simulink model "tutorial_picooz_acquire_extmode"  (R2025b)
settings: Solver=FixedStepDiscrete  StartTime=0.0  StopTime=60  FixedStep=0.001  RelTol=1e-3  EnableMultiTasking=on
undefined symbols (not defined in the file or in its folder): A0, ADC, D10, H0, Max, MaxPer, ms, ns, P1, P113, P59, Pin, PWM3_Trg1, Resol, us
libraries: MCHP_Blockset x8, simulink x5, dspsrcs4 x1, dspstat3 x1
(part 1 of 2)
settings Model: SimulationMode=external  ExtModeTrigDuration=20  Creator=Lubin Kerhuel  LastModifiedBy=Lubin Kerhuel
settings OptimizationCC: DefaultParameterBehavior=Inlined  DefaultUnderspecifiedDataType=single  EnhancedBackFolding=on  BooleansAsBitfields=on  PassReuseOutputArgsAs=Individual arguments  ZeroExternalMemoryAtStartup=off  ZeroInternalMemoryAtStartup=off  OptimizeBlockOrder=speed  DifferentSizesBufferReuse=on  EfficientTunableParamExpr=on
settings DebuggingCC: ParameterTunabilityLossMsg=error
settings HardwareCC: ProdBitPerPointer=32.0  ProdBitPerSizeT=32.0  ProdBitPerPtrDiffT=32.0  ProdLargestAtomicInteger=Long  ProdWordSize=32.0  ProdLongLongMode=on  ProdHWDeviceType=Generic->Custom
settings ModelReferenceCC: ModelReferenceNumInstancesAllowed=Single
settings SFSimCC: MATLABDynamicMemAlloc=off
settings RTWCC: SystemTargetFile=MCHP_dsPIC33A_noTMF_stf.tlc  TLCOptions="-aExtModeXCPClassicInterface=0  -aCreateExtModeTypes=1 -aExtModeXCPSimulationTimeInTicks=1"  TemplateMakefile=MCHP_dsPIC33A.tmf  Toolchain=MPLAB XC-DSC - v4.00_TC1 for dsPIC DSCs (Microchip)  BuildConfiguration=Specify  Description=Microchip Embedded Target dsPIC33A no TMF (real-time)
settings CodeAppCC: ForceParamTrailComments=on  IgnoreCustomStorageClasses=off  MaxIdLength=255.0  OperatorAnnotations=on  SimulinkDataObjDesc=on  SFDataObjDesc=on  InsertBlockDesc=on
settings STFCustomTargetCC: SystemTargetFile=MCHP_dsPIC33A_noTMF_stf.tlc  TargetLangStandard=C99 (ISO)  MultiwordLength=256.0  ConcurrentExecutionCompliant=off  CombineOutputUpdateFcns=on  CombineSignalStateStructs=on  ERTCustomFileBanners=on  SupportContinuousTime=off  RemoveResetFunc=on  MATLABClassNameForMDSCustomization=Simulink.SoftwareTarget.ERTCustomization  GRTInterface=off  UseToolchainInfoCompliant=on  MCHP_AUTO_FLASH=off  LINKER_SCRIPT=p33AK512MPS512.gld  EXTMODE_DATA_UPLOAD=on  RTWGenSettings_txt="s.RefMasterBlk='PICOOZ_OL_ExtMode_Curiosity_dsPIC33AK512MPS512/Microchip Master';s.ChipIdN='[33  512  512]';s.ChipIdL1='AK';s.ChipIdL2='MPS';s.ChipIdL3=' ';s.arch3='33A';s.ChipId='33AK512MPS512';s.Arch='8';s.bitFieldsSFR='4';s.ChipRAM='32768';s.ChipRAM_XBegin='16384';s.ChipRAM_dma='[-1 -1]';s.FuseConfigTxt='#pragma config FICD_JTAGEN = OFF\\\\n';s.TimeStep_Timer='-1';s.TimeStep_SyncADC='1';s.ADPCFG='0';s.ANSEL_Exist='1';s.ANSEL='[-1 -1 -1 -1 -1 -1 -1 -1 -1 -1 -1]';s.TRIS='[65535  65535    255  65535     -1     -1     -1  65535     -1     -1     -1     -1     -1     -1     -1     -1     -1     -1     -1     -1     -1     -1     -1     -1     -1     -1     -1     -1     -1     -1     -1     -1     -1     -1     -1     -1     -1     -1     -1     -1     -1     -1     -1     -1     -1     -1     -1     -1     -1     -1     -1     -1     -1     -1     -1     -1     -1]';s.RPOR='[-1  -1  -1  -1  -1  -1  -1  -1  -1  -1  -1  -1  -1  -1  -1  -1  -1  -1  -1  -1  -1  -1  -1  -1  -1  -1  -1  -1  19  -1  -1  -1  -1  -1  -1  -1]';s.RPINR='[-1  -1  -1  -1  -1  -1  -1  -1  -1  -1  -1  -1  -1  59  -1  -1  -1  -1  -1  -1  -1  -1  -1  -1  -1  -1  -1  -1]';s.LATSET='[-1 -1 -1 -1 -1 -1 -1 -1 -1 -1 -1 -1 -1 -1 -1 -1 -1 -1 -1 -1 -1 -1 -1 -1 -1 -1 -1 -1 -1 -1 -1 -1 -1 -1 -1 -1 -1 -1 -1 -1 -1 -1 -1 -1 -1 -1 -1 -1 -1 -1 -1 -1 -1 -1 -1 -1 -1]';s.LATCLR='[-1 -1 -1 -1 -1 -1 -1 -1 -1 -1 -1 -1 -1 -1 -1 -1 -1 -1 -1 -1 -1 -1 -1 -1 -1 -1 -1 -1 -1 -1 -1 -1 -1 -1 -1 -1 -1 -1 -1 -1 -1 -1 -1 -1 -1 -1 -1 -1 -1 -1 -1 -1 -1 -1 -1 -1 -1]';s.ODC='[-1 -1 -1 -1 -1 -1 -1 -1 -1 -1 -1 -1 -1 -1 -1 -1 -1 -1 -1 -1 -1 -1 -1 -1 -1 -1 -1 -1 -1 -1 -1 -1 -1 -1 -1 -1 -1 -1 -1 -1 -1 -1 -1 -1 -1 -1 -1 -1 -1 -1 -1 -1 -1 -1 -1 -1 -1]';s.CNPU='[-1 -1 -1 -1 -1 -1 -1 -1 -1 -1 -1 -1 -1 -1 -1 -1 -1 -1 -1 -1 -1 -1 -1 -1 -1 -1 -1 -1 -1 -1 -1 -1 -1 -1 -1 -1 -1 -1 -1 -1 -1 -1 -1 -1 -1 -1 -1 -1 -1 -1 -1 -1 -1 -1 -1 -1 -1]';s.CNPD='[-1 -1 -1 -1 -1 -1 -1 -1 -1 -1 -1 -1 -1 -1 -1 -1 -1 -1 -1 -1 -1 -1 -1 -1 -1 -1 -1 -1 -1 -1 -1 -1 -1 -1 -1 -1 -1 -1 -1 -1 -1 -1 -1 -1 -1 -1 -1 -1 -1 -1 -1 -1 -1 -1 -1 -1 -1]';s.PortConfigTxt=' ';s.CLKDIV='0';s.PLLFBD='-1';s.PLLDIV='16815713';s.QUARTZ='8000000';s.SWITCH_OSC='16386';s.PLLRNG='-1';s.MASTER_BusyFlag='-1';s.POWERSAVE='0';s.MIPS='200000000';s.FLASH_ECC='0';s.PBxDIV='[-1]';s.CLKx_INTDIV='[-1 -1 -1 -1  0  1  0  0  0 -1 -1  0  0]';s.CLKx_FRACDIV='[-1   -1   -1   -1    0  256    0    0    0   -1   -1    0    0]';s.AN_type2='1';s.ACLKCON_reg='-1';s.nTIMERS='3';s.nSCCP='9';s.DOS_04094_cpu_33a_v1_dspic33a='1';s.DOS_04436_perseus_dspic33a='0';s.DOS_04928_gpio_ports_upb_v2_dspic33a='1';s.DOS_02672_math_progcrc_upb_v1_dspic33a='1';s.DOS_04993_sec_32bit_cp_upb_v1_dspic33a='1';s.DOS_03459_adc_pc_ctrl_upb_v2_dspic33a='0';s.DOS_04302_pwm_pc_upb_v3_dspic33a='0';s.DOS_03076_uart_protocol_upb_v1_dspic33a='1';s.DOS_01482_spi_i2s_upb_v1_dspic33a='1';s.DOS_05155_i2c_upb_v4_dspic33a='1';s.DOS_02359_sent_j2716_upb_v1_dspic33a='1';s.DOS_05177_qei_32b_upb_v2_dspic33a='1';s.DOS_01512_ccp_mccp_upb_v1_dspic33a='1';s.DOS_03496_dac_pdm_nbit_upb_v2_dspic33a='0';s.DOS_02673_tmr_classa_upb_v1_dspic33a='1';s.DOS_04776_perf_mon_upb_v1_dspic33a='1';s.DOS_03680_pfm_pbu_33a_upb_v1_dspic33a='1';s.DOS_04649_sec_pac_upb_v0_dspic33a='0';s.DOS_03966_io_integrity_monitor_upb_v1_dspic33a='1';s.DOS_04641_biss_master_upb_v1_dspic33a='1';s.DOS_04077_dma_upb_v1_dspic33a='1';s.DOS_04549_nvm_ctrl_32bit_upb_v1_dspic33a='1';s.DOS_04449_clk_cru_33a_upb_v1_dspic33a='1';s.DOS_03850_clk_monitor_upb_v1_dspic33a='1';s.DOS_04342_osc_rc8mhz_ctrl_upb_v4_dspic33a='1';s.DOS_04650_wdt_upb_v4_dspic33a='1';s.DOS_05178_ptg_pc_upb_v2_dspic33a='1';s.DOS_04181_data_ram_ctrl_upb_v1_dspic33a='1';s.DOS_04735_wdt_dmt_upb_v6_dspic33a='1';s.DOS_01577_cla_clc_upb_v1_dspic33a='1';s.DOS_03516_pwr_sib_upb_v3_dspic33a='0';s.DOS_03495_amp_pad_opamp_ctrl_upb_v2_dspic33a='1';s.DOS_05830_blueRidge_dspic33a='0';s.DOS_05972_adc_12b_upb_v3_itc_dspic33a='0';s.DOS_05404_adc_pc_ctrl_upb_v3_dspic33a='1';s.DOS_05226_pwm_pc_upb_v4_dspic33a='1';s.DOS_05514_qei_32b_upb_v3_dspic33a='0';s.DOS_05431_dac_pdm_nbit_upb_v3_dspic33a='1';s.DOS_05828_pfm_pbu_33a_upb_v2_dspic33a='0';s.DOS_05765_math_rdc_upb_v1_32bit='0';s.DOS_05908_math_cic_upb_v2_32bit='0';s.DOS_05801_dma_upb_v2_dspic33a='0';s.DOS_05461_pwr_sib_upb_v4_dspic33a='1';s.DOS_05420_amp_vref_ctl_upb_v1_dspic33a='1';s.DOS_05592_pwr_monitor_sib_upb_v1='0';s.DOS_05924_bus_dual_die_upb_v2='0';s.DOS_06048_sec_cam_v3_dspic33a='0';s.DOS_05922_i3c_upb_v1_32bit='0';s.DOS_06006_adc_soft_code_seq_v2_dspic33a='0';s.DOS_05442_icd_trace_33a_v1_dspic33a='0';s.DOS_04537_can_fd_upb_v3_dspic33a='1';s.DOS_05308_pegasus_dspic33a='1';s.DOS_02976_adc_12b_upb_v2_dspic33a='1';s.DOS_05226_apwm_pc_upb_v4_dspic33a='1';s.DOS_04649_sec_pac_upb_v1_dspic33a='1';s.DOS_05346_sec_cam_v2_dspic33a='1';s.DOS_03267_adc_soft_code_seq_v1_dspic33a='1';s.DOS_05557_serpens_dspic33a='0';s.DOS_05972_adc_12b_upb_v3_adc_dspic33a='0';s.DOS_03681_bmx_33a_upb_v1_dspic33a='0';s.DOS_02050_tmr_rtcc_upb_v1_dspic33a='0';s.DOS_04649_sec_pac_upb_serpens_dspic33a='0';s.DOS_05692_pwr_sib_upb_v5_dspic33a='0';s.DOS_06006_adc_soft_code_seq_v2_adc_dspic33a='0';s.DOS_02551_cpu_16bit_v7='0';s.DOS_01520_wdt_dmt_upb_v1_16bit='0';s.DOS_02359a_sent_j2716_upb_v1='0';s.DOS_02672_math_progcrc_upb_v1_16bit='0';s.DOS_01577_cla_clc_upb_v1='0';s.DOS_02915_ecc_v2='0';s.DOS_02673_tmr_classa_upb_v1_16bit='0';s.DOS_01494_qei_32b_upb_v1_16bit='0';s.DOS_02472_ppi_pmp16_upb_v1_16bit='0';s.DOS_01441_i2c_upb_v1_16bit_TLAH='0';s.DOS_03076_uart_protocol_upb_v1_16bit='0';s.DOS_01482='0';s.DOS_01483_pwm_16bit='0';s.DOS_02949_WACG='0';s.DOS_02316_nvm_ctrl_v1_16bit='0';s.DOS_03349_amp_pad_opamp_ctrl_upb_v1='0';s.DOS_02653_afe_current_bias_ctrl_upb_v1_16bit='0';s.DOS_01459_ptg_pc_upb_v1_16bit='0';s.DOS_01512_ccp_mccp_upb_v1_16bit='0';s.DOS_02519_dma_sfr_16bit_v2='0';s.DOS_02508c11='0';s.DOS_02475_dac_pdm_nbit_upb_v1_16bit='0';s.DOS_02467_gpio_upb_v1_16bit='0';s.DOS_00805_rst_integration_v4='0';s.DOS_02659_clk_sib_v12='0';s.DOS_02237_osc_dco_ctrl_upb_v1_16bit='0';s.DOS_02674_wdt_upb_v1_16bit='0';s.DOS_01407='0';s.DOS_03247_CAN_FD_UPB_V2_16_bit='0';s.DOS_03994_WAC07='0';s.DOS_02552_msi_upb_v1_Master='0';s.DOS_03667_pwm_pc_upb_v2_16bit='0';s.DOS_04180_drm_ctrl_ecc_v1='0';s.DOS_03431_STX03='0';s.DOS_03516_pwr_sib_upb_v3='0';s.DOS_02552_msi_upb_v1_Slave='0';s.DOS_04621_amp_pga_ctrl_upb_v3='0';s.DOS_02497_WACV='0';s.DOS_02593_amp_pga_ctrl_pb_v2_16bit='0';s.DOS_01461_afe_ctmu_con_upb_v1_16bit='0';s.DOS_02497_WACA='0';s.DOS_02478_uart_irda_upb_v1_16bit='0';s.DOS_00929='0';s.DOS_01198='0';s.DOS_03029_WACH='0';s.DOS_01483_apwm_16bit='0';s.DOS_04797_WAC0A='0';s.DOS_04884_WAC0B='0';s.DOS_04797_WAC09='0';s.DOS_03662_WACU='0';s.DOS_00794='0';s.DOS_00931='0';s.DOS_00932='0';s.DOS_00942='0';s.DOS_00938='0';s.DOS_00996='0';s.DOS_00997='0';s.DOS_00998='0';s.DOS_00209='0';s.DOS_01555_adc='0';s.DOS_01293='0';s.DOS_00828='0';s.DOS_01116='0';s.DOS_01017_RPORx='0';s.DOS_01017_RPINRx='0';s.DOS_01555_nvm_tsmc18_v2_16bit='0';s.DOS_00804='0';s.DOS_00826='0';s.DOS_01555_TLAK_PMDx='0';s.DOS_01555_TLAK_INT_='0';s.DOS_00933='0';s.DOS_01555='0';s.DOS_01555_ptg='0';s.DOS_00958='0';s.DOS_01117_PORTx='0';s.DOS_00999='0';s.DOS_01041='0';s.DOS_00892='0';s.DOS_01287_TLAC_PMDx='0';s.DOS_01287_TLAC_INT_='0';s.DOS_01424='0';s.DOS_01332='0';s.DOS_01468_PMBA_current_source='0';s.DOS_02291_PGA='0';s.DOS_01467_Comparator='0';s.DOS_01498_TLAY='0';s.DOS_00993_PLL_120MHz='0';s.DOS_01332_ptg_pc_v1='0';s.DOS_00958_pwm_TLAY='0';s.TLAY_IOPorts='0';s.DOS_00929q='0';s.DOS_02415_spi_v5='0';s.DOS_RPINRx_16bit_2='0';s.DOS_01497_TLAH_PMDx='0';s.DOS_02550_TLAL_INT='0';s.DOS_00958_pwm_TLAH='0';s.DOS_01287_TLAH_INT_='0';s.DOS_01113='0';s.DOS_01017_PMDx='0';s.DOS_00927='0';s.DOS_01080='0';s.DOS_00794_cpu_16bit_v3='0';s.DOS_02192_TLCD_PMDx='0';s.DOS_02192_TLCD_INT_='0';s.DOS_02192_cmp='0';s.DOS_00958_pwm_TLCD='0';s.DOS_02192_PORTx_TLCD='0';s.DOS_00936='0';s.DOS_00995='0';s.DOS_00546='0';s.DOS_00474='0';s.DOS_02481_WACP_Config='0';s.DOS_03088_pfm_cache_ocp_v2_WACK='0';s.DOS_02819_pfm_ctrl_32bit_upb_v2='0';s.DOS_02674_wdt_upb_v1_32bit='0';s.DOS_01520_wdt_dmt_upb_v1='0';s.DOS_02869_icd_jtag_bvci_upb_v2='0';s.DOS_02823_WACJ_clk_cru_upb_v2='0';s.DOS_02823_WACN_clk_cru_upb_v2='0';s.DOS_01423_RPINRx='0';s.DOS_02481_RPORx='0';s.DOS_02511_pwr_sib_upb_v1_32bit='0';s.DOS_02907_WACP_int_evic_v3='0';s.DOS_01500_dma_bvci_v2='0';s.DOS_02141_tmr_classa_pb_v2='0';s.DOS_02815_tmr_classb_upb_v1='0';s.DOS_00740_icap_pb_v1='0';s.DOS_00749_ocmp_pb_v1='0';s.DOS_01441_i2c_upb_v1_32bit='0';s.DOS_01329_spi_pb_v2='0';s.DOS_02478_uart_irda_upb_v1_32bit='0';s.DOS_01477_pwm_mc_upb_v1='0';s.DOS_01494_qei_32b_upb_v1='0';s.DOS_03554_cmp_control_upb_v2_32bit='0';s.DOS_01445_dac_nbit__control_upb_v1_32bit='0';s.DOS_01461_afe_ctmu_con_upb_v1='0';s.DOS_01577_cla_clc_upb_v1_32bit='0';s.DOS_02467_gpio_ports_upb_v1='0';s.DOS_02508_WACP_adc_sar_ctrl_upb_v1='0';s.DOS_01261_tmr_rtcc_WACJ_K_N_P_pb_v2='0';s.DOS_EIP_00136_ssx_v1='0';s.DOS_02481_WACK_MC_Config='0';s.DOS_02907_WACN_GP_int_evic_v3='0';s.DOS_02508_adc_sar_ctrl_upb_v1_PIC32MK='0';s.DOS_01261_tmr_rtcc_pb_v2='0';s.DOS_01475_lpwr_deep_sleep_ctrl_v2='0';s.DOS_02907_WACN_MC_int_evic_v3='0';s.DOS_03247_can_fd_upb_v2_pic32mk='0';s.DOS_02907_WACK_MC_int_evic_v3='0';s.DOS_02514_dfm_strl_sst_upb_v1='0';s.DOS_02472_ppi_pmp16_upb_v1='0';s.DOS_02813a_usb_otgcore_pb_v3='0';s.DOS_02481_WACJ_MC_Config='0';s.DOS_02569_pfm_cache_ocp_v1='0';s.DOS_02481_WACJ_MC_int_evic_v3='0';s.DOS_01459_ptg_pc_upb_v1_SIC='0';s.DOS_01427_cmp_control_upb_v1_32bit='0';s.DOS_01152_can_bvci_v1='0';s.DOS_02787_WACD_Config='0';s.DOS_00800_dac_4bit_ctrl_pb_v1='0';s.DOS_01539_icd_jtag_pb_v2='0';s.DOS_02823_clk_cru_upb_v2='0';s.DOS_01423_RPORx='0';s.DOS_02907_WACD_int_evic_v3='0';s.DOS_00734_uart_irda_pb_v1='0';s.DOS_00687_tmr_classa_pb_v1='0';s.DOS_00745_tmr_classb_pb_v1='0';s.DOS_02508_adc_sar_ctrl_upb_v1='0';s.DOS_00866_cmp_control_pb_v2='0';s.DOS_01114_eth_bvci_v1='0';s.DOS_02831_usb_clk_rst_v2='0';s.DOS_01643_pfm_cache_ahb_v2='0';s.DOS_EIP_00206r5_sqi_v2='0';s.DOS_EIP_00124_usb_hs_otgcore_v1='0';s.DOS_EIP_00218_math_rng_ahbs_v2='0';s.DOS_EIP_00109_ebi_v1='0';s.DOS_EIP_00158_crypto_v1='0';s.UART_TX_IMPLEMENTATION='[2]';s.UART_RX_IMPLEMENTATION='[2]';s.UART_TX_DMACHANNEL='[0]';s.UART_HALF_DUPLEX_MODE='[0]';s.UART_TX_THREAD_PROTECTION='[9]';"  HOST_PLATFORM=PC  PIC_REF=33AK512MPS512  OBJDUMP=xc-dsc-objdump  BIN2HEX=xc-dsc-bin2hex  MCHP_MULTITHREAD_COMPILATION=on  TIMER_START="[0  0  0  0]"  LinkWithMaster=off  GCCPATH=C:/PROGRA~1/MICROC~1/xc-dsc/V44CDE~1.00_/bin  AssemblyListing=off  AR1=xc-dsc-ar  OPTIM_GCC=-O2 -fno-short-double -mno-eds-warn -mconst-in-data -mlarge-data -mlarge-aggregate -g -Wa,--reorder  LDFLAGS='--report-mem,-Map=$(PRODUCT_NAME).map,-cref,-lq-dsp'  ProduceHexOutput=off  TIMER_PERIOD="[0      0      0  65535]"  GCC1=xc-dsc-gcc.exe  TIMER_PRESCALER="[-1 -1 -1  3 -1 -1 -1 -1 -1 -1 -1 -1]"  MCHP_XCP_MemoryBlockParameters=[-1 8]
settings ERTTargetCC: ExtMode=on  ExtModeTransport=1.0  ExtModeStaticAlloc=on  ExtModeMaxTrigDuration=20.0  ExtModeStaticAllocSize=2048.0  ExtModeMexFile=ext_xcp  ExtModeMexArgs=1 27 460800 './PICOOZ_OL_ExtMode_Curiosity_dsPIC33AK512MPS512.X/PICOOZ_OL_ExtMode_Curiosity_dsPIC33AK512MPS512.elf'  ExtModeIntrfLevel=Level2 - Open  ERTSrcFileBannerTemplate=MCHP_dsPIC_code_template.cgt  ERTHdrFileBannerTemplate=MCHP_dsPIC_code_template.cgt  ERTDataSrcFileTemplate=MCHP_dsPIC_code_template.cgt  ERTDataHdrFileTemplate=MCHP_dsPIC_code_template.cgt  ERTCustomFileTemplate=MCHP_main.tlc  MaxLineWidth=110.0  TargetLangStandard=C99 (ISO)  ParMdlRefBuildCompliant=off  CompOptLevelCompliant=off  ConcurrentExecutionCompliant=off  CombineSignalStateStructs=on  SupportNonInlinedSFcns=on  ModelStepFunctionPrototypeControlCompliant=off  CPPClassGenCompliant=off

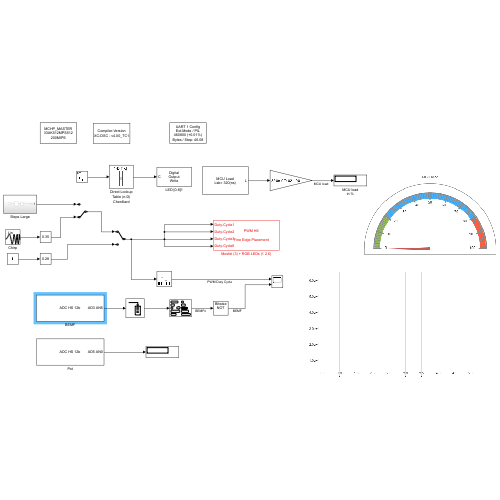
[thumbnail: Simulink's stored preview of the top-level diagram]
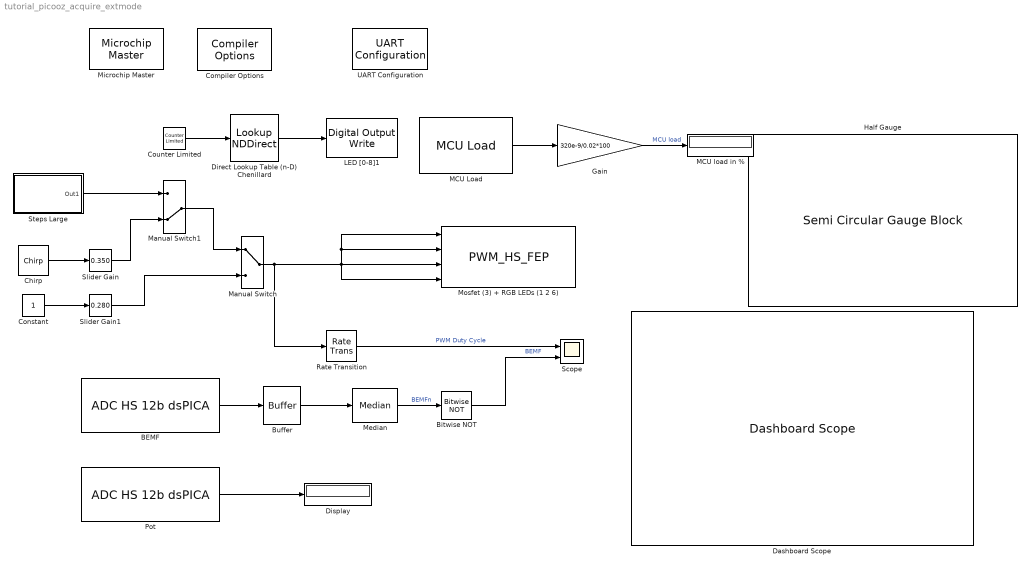
== system tutorial_picooz_acquire_extmode ==
  BEMF : MCHP_Blockset/Analog IO/ADC HS 12b dsPICA  ADCREF=ADC 1 and ADC 2  ADC1_refChannel=Not used  ADC2_refChannel=Not used  ADC3_refChannel=0 (highest priority)  ADC4_refChannel=Not used  ADC5_refChannel=Not used  CALRATE=once at startup  VREF_RNG=3.0V to 3.6V  BUFEN=off  info=0  SampleTime=.001  MCHP_PORT={ADC1_seq0.0}{ADC1A2}15:2:A2;{ADC2_seq0.0}{ADC2B0}15:2:B0;{ADC1_seq1.0}{ADC1A2}15:2:A2;{ADC2_seq1.0}{ADC2B0}15:2:B0;{ADC1_seq2.0}{ADC1A2}15:2:A2;{ADC2_seq2.0}{ADC2B0}15:2:B0;{ADC1_seq3.0}{ADC1A2}15:2:A2;{ADC2_seq3.0}{ADC2B0}15:2:B0;{ADC1_seq4.0}{ADC1A2}15:2:A2;{ADC2_seq4.0}{ADC2B0}15:2:B0;{ADC1_seq5.0}{ADC1A2}15:2:A2;{ADC2_seq5.0}{ADC2B0}15:2:B0;{ADC1_seq0.0}{ADC1A2}15:2:A2;{ADC2_seq0.0}{ADC2B0}15:2:B0;{ADC1_seq1.0}{ADC1A2}15:2:A2;{ADC2_seq1.0}{ADC2B0}15:2:B0;{ADC1_seq2.0}{ADC1A2}15:2:A2;{ADC2_seq2.0}{ADC2B0}15:2:B0;{ADC1_seq3.0}{ADC1A2}15:2:A2;{ADC2_seq3.0}{ADC2B0}15:2:B0;{ADC1_seq4.0}{ADC1A2}15:2:A2;{ADC2_seq4.0}{ADC2B0}15:2:B0;{ADC1_seq5.0}{ADC1A2}15:2:A2;{ADC2_seq5.0}{ADC2B0}15:2:B0;  MCHP_MASTERLINK=PICOOZ_OL_ExtMode_Curiosity_dsPIC33AK512MPS512/Microchip Master  MCHP_CRC=27486782  ADC_Synchronisation=Triggered by custom source  ADC_Trig_TXT=PWM3_Trg1  ADC_TrigTimeStep=on  TrigSource_seq0_TXT=PWM3 adc trig 1  SampleTime_seq0_Tad_TXT="4.5 Tad  = 56.2ns  -  Rin < 5.2 kOhm"  ADC1_seq0_TXT=AD1 AN0 / A2 / Pin[25]  ADC1_seq0_align=Left aligned  ADC1_seq0_overSampling=x1 (12 bits)  ADC2_seq0_TXT=AD2 AN0 / B0 / Pin[41]  ADC2_seq0_align=Right aligned  ADC2_seq0_overSampling=x1 (12 bits)  ADC3_seq0_TXT=AD3 AN5 / A0 / Pin[4]  ADC3_seq0_align=Left aligned  ADC3_seq0_overSampling=x256 (16 bits)  ADC4_seq0_TXT=AD4 AN0 / B4 / Pin[57]  ADC4_seq0_align=Left aligned  ADC4_seq0_overSampling=x1 (12 bits)  ADC5_seq0_TXT=AD5 AN0 / A7 / Pin[5]  ADC5_seq0_align=Left aligned  ADC5_seq0_overSampling=x1 (12 bits)  ADC1_seq0_1_TXT=Not Used  ADC1_seq0_1_align=Right aligned  ADC1_seq0_1_overSampling=x1 (12 bits)  ADC2_seq0_1_TXT=Not Used  ADC2_seq0_1_align=Right aligned  ADC2_seq0_1_overSampling=x1 (12 bits)  ADC3_seq0_1_TXT=Not Used  ADC3_seq0_1_align=Right aligned  ADC3_seq0_1_overSampling=x1 (12 bits)  ADC4_seq0_1_TXT=Not Used  ADC4_seq0_1_align=Right aligned  ADC4_seq0_1_overSampling=x1 (12 bits)  ADC5_seq0_1_TXT=Not Used  ADC5_seq0_1_align=Right aligned  ADC5_seq0_1_overSampling=x1 (12 bits)  ADC1_seq0_2_TXT=Not Used  ADC1_seq0_2_align=Right aligned  ADC1_seq0_2_overSampling=x1 (12 bits)  ADC2_seq0_2_TXT=Not Used  ADC2_seq0_2_align=Right aligned  ADC2_seq0_2_overSampling=x1 (12 bits)  ADC3_seq0_2_TXT=Not Used  ADC3_seq0_2_align=Right aligned  ADC3_seq0_2_overSampling=x1 (12 bits)  ADC4_seq0_2_TXT=Not Used  ADC4_seq0_2_align=Right aligned  ADC4_seq0_2_overSampling=x1 (12 bits)  ADC5_seq0_2_TXT=Not Used  ADC5_seq0_2_align=Right aligned  ADC5_seq0_2_overSampling=x1 (12 bits)  ADC1_seq0_3_TXT=Not Used  ADC1_seq0_3_align=Right aligned  ADC1_seq0_3_overSampling=x1 (12 bits)  ADC2_seq0_3_TXT=Not Used  ADC2_seq0_3_align=Right aligned  ADC2_seq0_3_overSampling=x1 (12 bits)  ADC3_seq0_3_TXT=Not Used  ADC3_seq0_3_align=Right aligned  ADC3_seq0_3_overSampling=x1 (12 bits)  ADC4_seq0_3_TXT=Not Used  ADC4_seq0_3_align=Right aligned  ADC4_seq0_3_overSampling=x1 (12 bits)  ADC5_seq0_3_TXT=Not Used  ADC5_seq0_3_align=Right aligned  ADC5_seq0_3_overSampling=x1 (12 bits)  ADC1_seq0_4_TXT=Not Used  ADC1_seq0_4_align=Right aligned  ADC1_seq0_4_overSampling=x1 (12 bits)  ADC2_seq0_4_TXT=Not Used  ADC2_seq0_4_align=Right aligned  ADC2_seq0_4_overSampling=x1 (12 bits)  ADC3_seq0_4_TXT=Not Used  ADC3_seq0_4_align=Right aligned  ADC3_seq0_4_overSampling=x1 (12 bits)  ADC4_seq0_4_TXT=Not Used  ADC4_seq0_4_align=Right aligned  ADC4_seq0_4_overSampling=x1 (12 bits)  ADC5_seq0_4_TXT=Not Used  ADC5_seq0_4_align=Right aligned  ADC5_seq0_4_overSampling=x1 (12 bits)  ADC1_seq0_5_TXT=Not Used  ADC1_seq0_5_align=Right aligned  ADC1_seq0_5_overSampling=x1 (12 bits)  ADC2_seq0_5_TXT=Not Used  ADC2_seq0_5_align=Right aligned  ADC2_seq0_5_overSampling=x1 (12 bits)  ADC3_seq0_5_TXT=Not Used  ADC3_seq0_5_align=Right aligned  ADC3_seq0_5_overSampling=x1 (12 bits)  ADC4_seq0_5_TXT=Not Used  ADC4_seq0_5_align=Right aligned  ADC4_seq0_5_overSampling=x1 (12 bits)  ADC5_seq0_5_TXT=Not Used  ADC5_seq0_5_align=Right aligned  ADC5_seq0_5_overSampling=x1 (12 bits)  ADC_TRG2_ACCBRST_seq0=Burst - not interruptible  ADC1_NINSEL_seq0_TXT=Vss - single ended (unsigned)  ADC2_NINSEL_seq0_TXT=Vss - single ended (unsigned)  ADC3_NINSEL_seq0_TXT=Vss - single ended (unsigned)  ADC4_NINSEL_seq0_TXT=Vss - single ended (unsigned)  ADC5_NINSEL_seq0_TXT=Vss - single ended (unsigned)  TrigTimeStep_seq0=on  info_seq0=0  TrigSource_seq1_TXT=PWM1 adc trig 1  SampleTime_seq1_Tad_TXT="4.5 Tad  = 56.2ns  -  Rin < 5.2 kOhm"  ADC1_seq1_TXT=AD1 AN0 / A2 / Pin[25]  ADC1_seq1_align=Left aligned  ADC1_seq1_overSampling=x1 (12 bits)  ADC2_seq1_TXT=AD2 AN0 / B0 / Pin[41]  ADC2_seq1_align=Right aligned  ADC2_seq1_overSampling=x1 (12 bits)  ADC3_seq1_TXT=Not Used  ADC3_seq1_align=Left aligned  ADC3_seq1_overSampling=x1 (12 bits)  ADC4_seq1_TXT=AD4 AN0 / B4 / Pin[57]  ADC4_seq1_align=Left aligned  ADC4_seq1_overSampling=x1 (12 bits)  ADC5_seq1_TXT=AD5 AN0 / A7 / Pin[5]  ADC5_seq1_align=Left aligned  ADC5_seq1_overSampling=x1 (12 bits)  ADC1_seq1_1_TXT=Not Used  ADC1_seq1_1_align=Right aligned  ADC1_seq1_1_overSampling=x1 (12 bits)  ADC2_seq1_1_TXT=Not Used  ADC2_seq1_1_align=Right aligned  ADC2_seq1_1_overSampling=x1 (12 bits)  ADC3_seq1_1_TXT=Not Used  ADC3_seq1_1_align=Right aligned  ADC3_seq1_1_overSampling=x1 (12 bits)  ADC4_seq1_1_TXT=Not Used  ADC4_seq1_1_align=Right aligned  ADC4_seq1_1_overSampling=x1 (12 bits)  ADC5_seq1_1_TXT=Not Used  ADC5_seq1_1_align=Right aligned  ADC5_seq1_1_overSampling=x1 (12 bits)  ADC1_seq1_2_TXT=Not Used  ADC1_seq1_2_align=Right aligned  ADC1_seq1_2_overSampling=x1 (12 bits)  ADC2_seq1_2_TXT=Not Used  ADC2_seq1_2_align=Right aligned  ADC2_seq1_2_overSampling=x1 (12 bits)  ADC3_seq1_2_TXT=Not Used  ADC3_seq1_2_align=Right aligned  ADC3_seq1_2_overSampling=x1 (12 bits)  ADC4_seq1_2_TXT=Not Used  ADC4_seq1_2_align=Right aligned  ADC4_seq1_2_overSampling=x1 (12 bits)  ADC5_seq1_2_TXT=Not Used  ADC5_seq1_2_align=Right aligned  ADC5_seq1_2_overSampling=x1 (12 bits)  ADC1_seq1_3_TXT=Not Used  ADC1_seq1_3_align=Right aligned  ADC1_seq1_3_overSampling=x1 (12 bits)  ADC2_seq1_3_TXT=Not Used  ADC2_seq1_3_align=Right aligned  ADC2_seq1_3_overSampling=x1 (12 bits)  ADC3_seq1_3_TXT=Not Used  ADC3_seq1_3_align=Right aligned  ADC3_seq1_3_overSampling=x1 (12 bits)  ADC4_seq1_3_TXT=Not Used  ADC4_seq1_3_align=Right aligned  ADC4_seq1_3_overSampling=x1 (12 bits)  ADC5_seq1_3_TXT=Not Used  ADC5_seq1_3_align=Right aligned  ADC5_seq1_3_overSampling=x1 (12 bits)  ADC1_seq1_4_TXT=Not Used  ADC1_seq1_4_align=Right aligned  ADC1_seq1_4_overSampling=x1 (12 bits)  ADC2_seq1_4_TXT=Not Used  ADC2_seq1_4_align=Right aligned  ADC2_seq1_4_overSampling=x1 (12 bits)  ADC3_seq1_4_TXT=Not Used  ADC3_seq1_4_align=Right aligned  ADC3_seq1_4_overSampling=x1 (12 bits)  ADC4_seq1_4_TXT=Not Used  ADC4_seq1_4_align=Right aligned  ADC4_seq1_4_overSampling=x1 (12 bits)  ADC5_seq1_4_TXT=Not Used  ADC5_seq1_4_align=Right aligned  ADC5_seq1_4_overSampling=x1 (12 bits)  ADC1_seq1_5_TXT=Not Used  ADC1_seq1_5_align=Right aligned  ADC1_seq1_5_overSampling=x1 (12 bits)  ADC2_seq1_5_TXT=Not Used  ADC2_seq1_5_align=Right aligned  ADC2_seq1_5_overSampling=x1 (12 bits)  ADC3_seq1_5_TXT=Not Used  ADC3_seq1_5_align=Right aligned  ADC3_seq1_5_overSampling=x1 (12 bits)  ADC4_seq1_5_TXT=Not Used  ADC4_seq1_5_align=Right aligned  ADC4_seq1_5_overSampling=x1 (12 bits)  ADC5_seq1_5_TXT=Not Used  ADC5_seq1_5_align=Right aligned  ADC5_seq1_5_overSampling=x1 (12 bits)  ADC_TRG2_ACCBRST_seq1=Burst - not interruptible  ADC1_NINSEL_seq1_TXT=Vss - single ended (unsigned)  ADC2_NINSEL_seq1_TXT=Vss - single ended (unsigned)  ADC3_NINSEL_seq1_TXT=Vss - single ended (unsigned)  ADC4_NINSEL_seq1_TXT=Vss - single ended (unsigned)  ADC5_NINSEL_seq1_TXT=Vss - single ended (unsigned)  TrigTimeStep_seq1=on  info_seq1=0  TrigSource_seq2_TXT=PWM1 adc trig 1  SampleTime_seq2_Tad_TXT="4.5 Tad  = 56.2ns  -  Rin < 5.2 kOhm"  ADC1_seq2_TXT=AD1 AN0 / A2 / Pin[25]  ADC1_seq2_align=Left aligned  ADC1_seq2_overSampling=x1 (12 bits)  ADC2_seq2_TXT=AD2 AN0 / B0 / Pin[41]  ADC2_seq2_align=Right aligned  ADC2_seq2_overSampling=x1 (12 bits)  ADC3_seq2_TXT=Not Used  ADC3_seq2_align=Left aligned  ADC3_seq2_overSampling=x1 (12 bits)  ADC4_seq2_TXT=AD4 AN0 / B4 / Pin[57]  ADC4_seq2_align=Left aligned  ADC4_seq2_overSampling=x1 (12 bits)  ADC5_seq2_TXT=AD5 AN0 / A7 / Pin[5]  ADC5_seq2_align=Left aligned  ADC5_seq2_overSampling=x1 (12 bits)  ADC1_seq2_1_TXT=Not Used  ADC1_seq2_1_align=Right aligned  ADC1_seq2_1_overSampling=x1 (12 bits)  ADC2_seq2_1_TXT=Not Used  ADC2_seq2_1_align=Right aligned  ADC2_seq2_1_overSampling=x1 (12 bits)  ADC3_seq2_1_TXT=Not Used  ADC3_seq2_1_align=Right aligned  ADC3_seq2_1_overSampling=x1 (12 bits)  ADC4_seq2_1_TXT=Not Used  ADC4_seq2_1_align=Right aligned  ADC4_seq2_1_overSampling=x1 (12 bits)  ADC5_seq2_1_TXT=Not Used  ADC5_seq2_1_align=Right aligned  ADC5_seq2_1_overSampling=x1 (12 bits)  ADC1_seq2_2_TXT=Not Used  ADC1_seq2_2_align=Right aligned  ADC1_seq2_2_overSampling=x1 (12 bits)  ADC2_seq2_2_TXT=Not Used  ADC2_seq2_2_align=Right aligned  ADC2_seq2_2_overSampling=x1 (12 bits)  ADC3_seq2_2_TXT=Not Used  ADC3_seq2_2_align=Right aligned  ADC3_seq2_2_overSampling=x1 (12 bits)  ADC4_seq2_2_TXT=Not Used  ADC4_seq2_2_align=Right aligned  ADC4_seq2_2_overSampling=x1 (12 bits)  ADC5_seq2_2_TXT=Not Used  ADC5_seq2_2_align=Right aligned  ADC5_seq2_2_overSampling=x1 (12 bits)  ADC1_seq2_3_TXT=Not Used  ADC1_seq2_3_align=Right aligned  ADC1_seq2_3_overSampling=x1 (12 bits)  ADC2_seq2_3_TXT=Not Used  ADC2_seq2_3_align=Right aligned  ADC2_seq2_3_overSampling=x1 (12 bits)  ADC3_seq2_3_TXT=Not Used  ADC3_seq2_3_align=Right aligned  ADC3_seq2_3_overSampling=x1 (12 bits)  ADC4_seq2_3_TXT=Not Used  ADC4_seq2_3_align=Right aligned  ADC4_seq2_3_overSampling=x1 (12 bits)  ADC5_seq2_3_TXT=Not Used  ADC5_seq2_3_align=Right aligned  ADC5_seq2_3_overSampling=x1 (12 bits)  ADC1_seq2_4_TXT=Not Used  ADC1_seq2_4_align=Right aligned  ADC1_seq2_4_overSampling=x1 (12 bits)  ADC2_seq2_4_TXT=Not Used  ADC2_seq2_4_align=Right aligned  ADC2_seq2_4_overSampling=x1 (12 bits)  ADC3_seq2_4_TXT=Not Used  ADC3_seq2_4_align=Right aligned  ADC3_seq2_4_overSampling=x1 (12 bits)  ADC4_seq2_4_TXT=Not Used  ADC4_seq2_4_align=Right aligned  ADC4_seq2_4_overSampling=x1 (12 bits)  ADC5_seq2_4_TXT=Not Used  ADC5_seq2_4_align=Right aligned  ADC5_seq2_4_overSampling=x1 (12 bits)  ADC1_seq2_5_TXT=Not Used  ADC1_seq2_5_align=Right aligned  ADC1_seq2_5_overSampling=x1 (12 bits)  ADC2_seq2_5_TXT=Not Used  ADC2_seq2_5_align=Right aligned  ADC2_seq2_5_overSampling=x1 (12 bits)  ADC3_seq2_5_TXT=Not Used  ADC3_seq2_5_align=Right aligned  ADC3_seq2_5_overSampling=x1 (12 bits)  ADC4_seq2_5_TXT=Not Used  ADC4_seq2_5_align=Right aligned  ADC4_seq2_5_overSampling=x1 (12 bits)  ADC5_seq2_5_TXT=Not Used  ADC5_seq2_5_align=Right aligned  ADC5_seq2_5_overSampling=x1 (12 bits)  ADC_TRG2_ACCBRST_seq2=Burst - not interruptible  ADC1_NINSEL_seq2_TXT=Vss - single ended (unsigned)  ADC2_NINSEL_seq2_TXT=Vss - single ended (unsigned)  ADC3_NINSEL_seq2_TXT=Vss - single ended (unsigned)  ADC4_NINSEL_seq2_TXT=Vss - single ended (unsigned)  ADC5_NINSEL_seq2_TXT=Vss - single ended (unsigned)  TrigTimeStep_seq2=on  info_seq2=0  TrigSource_seq3_TXT=PWM1 adc trig 1  SampleTime_seq3_Tad_TXT="4.5 Tad  = 56.2ns  -  Rin < 5.2 kOhm"  ADC1_seq3_TXT=AD1 AN0 / A2 / Pin[25]  ADC1_seq3_align=Left aligned  ADC1_seq3_overSampling=x1 (12 bits)  ADC2_seq3_TXT=AD2 AN0 / B0 / Pin[41]  ADC2_seq3_align=Right aligned  ADC2_seq3_overSampling=x1 (12 bits)  ADC3_seq3_TXT=Not Used  ADC3_seq3_align=Left aligned  ADC3_seq3_overSampling=x1 (12 bits)  ADC4_seq3_TXT=AD4 AN0 / B4 / Pin[57]  ADC4_seq3_align=Left aligned  ADC4_seq3_overSampling=x1 (12 bits)  ADC5_seq3_TXT=AD5 AN0 / A7 / Pin[5]  ADC5_seq3_align=Left aligned  ADC5_seq3_overSampling=x1 (12 bits)  ADC1_seq3_1_TXT=Not Used  ADC1_seq3_1_align=Right aligned  ADC1_seq3_1_overSampling=x1 (12 bits)  ADC2_seq3_1_TXT=Not Used  ADC2_seq3_1_align=Right aligned  ADC2_seq3_1_overSampling=x1 (12 bits)  ADC3_seq3_1_TXT=Not Used  ADC3_seq3_1_align=Right aligned  ADC3_seq3_1_overSampling=x1 (12 bits)  ADC4_seq3_1_TXT=Not Used  ADC4_seq3_1_align=Right aligned  ADC4_seq3_1_overSampling=x1 (12 bits)  ADC5_seq3_1_TXT=Not Used  ADC5_seq3_1_align=Right aligned  ADC5_seq3_1_overSampling=x1 (12 bits)  ADC1_seq3_2_TXT=Not Used  ADC1_seq3_2_align=Right aligned  ADC1_seq3_2_overSampling=x1 (12 bits)  ADC2_seq3_2_TXT=Not Used  ADC2_seq3_2_align=Right aligned  ADC2_seq3_2_overSampling=x1 (12 bits)  ADC3_seq3_2_TXT=Not Used  ADC3_seq3_2_align=Right aligned  ADC3_seq3_2_overSampling=x1 (12 bits)  ADC4_seq3_2_TXT=Not Used  ADC4_seq3_2_align=Right aligned  ADC4_seq3_2_overSampling=x1 (12 bits)  ADC5_seq3_2_TXT=Not Used  ADC5_seq3_2_align=Right aligned  ADC5_seq3_2_overSampling=x1 (12 bits)  ADC1_seq3_3_TXT=Not Used  ADC1_seq3_3_align=Right aligned  ADC1_seq3_3_overSampling=x1 (12 bits)  ADC2_seq3_3_TXT=Not Used  ADC2_seq3_3_align=Right aligned  ADC2_seq3_3_overSampling=x1 (12 bits)  ADC3_seq3_3_TXT=Not Used  ADC3_seq3_3_align=Right aligned  ADC3_seq3_3_overSampling=x1 (12 bits)  ADC4_seq3_3_TXT=Not Used  ADC4_seq3_3_align=Right aligned  ADC4_seq3_3_overSampling=x1 (12 bits)  ADC5_seq3_3_TXT=Not Used  ADC5_seq3_3_align=Right aligned  ADC5_seq3_3_overSampling=x1 (12 bits)  ADC1_seq3_4_TXT=Not Used  ADC1_seq3_4_align=Right aligned  ADC1_seq3_4_overSampling=x1 (12 bits)  ADC2_seq3_4_TXT=Not Used  ADC2_seq3_4_align=Right aligned  ADC2_seq3_4_overSampling=x1 (12 bits)  ADC3_seq3_4_TXT=Not Used  ADC3_seq3_4_align=Right aligned  ADC3_seq3_4_overSampling=x1 (12 bits)  ADC4_seq3_4_TXT=Not Used  ADC4_seq3_4_align=Right aligned  ADC4_seq3_4_overSampling=x1 (12 bits)  ADC5_seq3_4_TXT=Not Used  ADC5_seq3_4_align=Right aligned  ADC5_seq3_4_overSampling=x1 (12 bits)  ADC1_seq3_5_TXT=Not Used  ADC1_seq3_5_align=Right aligned  ADC1_seq3_5_overSampling=x1 (12 bits)  ADC2_seq3_5_TXT=Not Used  ADC2_seq3_5_align=Right aligned  ADC2_seq3_5_overSampling=x1 (12 bits)  ADC3_seq3_5_TXT=Not Used  ADC3_seq3_5_align=Right aligned  ADC3_seq3_5_overSampling=x1 (12 bits)  ADC4_seq3_5_TXT=Not Used  ADC4_seq3_5_align=Right aligned  ADC4_seq3_5_overSampling=x1 (12 bits)  ADC5_seq3_5_TXT=Not Used  ADC5_seq3_5_align=Right aligned  ADC5_seq3_5_overSampling=x1 (12 bits)  ADC_TRG2_ACCBRST_seq3=Burst - not interruptible  ADC1_NINSEL_seq3_TXT=Vss - single ended (unsigned)  ADC2_NINSEL_seq3_TXT=Vss - single ended (unsigned)  ADC3_NINSEL_seq3_TXT=Vss - single ended (unsigned)  ADC4_NINSEL_seq3_TXT=Vss - single ended (unsigned)  ADC5_NINSEL_seq3_TXT=Vss - single ended (unsigned)  TrigTimeStep_seq3=on  info_seq3=0  TrigSource_seq4_TXT=PWM1 adc trig 1  SampleTime_seq4_Tad_TXT="4.5 Tad  = 56.2ns  -  Rin < 5.2 kOhm"  ADC1_seq4_TXT=AD1 AN0 / A2 / Pin[25]  ADC1_seq4_align=Left aligned  ADC1_seq4_overSampling=x1 (12 bits)  ADC2_seq4_TXT=AD2 AN0 / B0 / Pin[41]  ADC2_seq4_align=Right aligned  ADC2_seq4_overSampling=x1 (12 bits)  ADC3_seq4_TXT=Not Used  ADC3_seq4_align=Left aligned  ADC3_seq4_overSampling=x1 (12 bits)  ADC4_seq4_TXT=AD4 AN0 / B4 / Pin[57]  ADC4_seq4_align=Left aligned  ADC4_seq4_overSampling=x1 (12 bits)  ADC5_seq4_TXT=AD5 AN0 / A7 / Pin[5]  ADC5_seq4_align=Left aligned  ADC5_seq4_overSampling=x1 (12 bits)  ADC1_seq4_1_TXT=Not Used  ADC1_seq4_1_align=Right aligned  ADC1_seq4_1_overSampling=x1 (12 bits)  ADC2_seq4_1_TXT=Not Used  ADC2_seq4_1_align=Right aligned  ADC2_seq4_1_overSampling=x1 (12 bits)  ADC3_seq4_1_TXT=Not Used  ADC3_seq4_1_align=Right aligned  ADC3_seq4_1_overSampling=x1 (12 bits)  ADC4_seq4_1_TXT=Not Used  ADC4_seq4_1_align=Right aligned  ADC4_seq4_1_overSampling=x1 (12 bits)  ADC5_seq4_1_TXT=Not Used  ADC5_seq4_1_align=Right aligned  ADC5_seq4_1_overSampling=x1 (12 bits)  ADC1_seq4_2_TXT=Not Used  ADC1_seq4_2_align=Right aligned  ADC1_seq4_2_overSampling=x1 (12 bits)  ADC2_seq4_2_TXT=Not Used  ADC2_seq4_2_align=Right aligned  ADC2_seq4_2_overSampling=x1 (12 bits)  ADC3_seq4_2_TXT=Not Used  ADC3_seq4_2_align=Right aligned  ADC3_seq4_2_overSampling=x1 (12 bits)  ADC4_seq4_2_TXT=Not Used  ADC4_seq4_2_align=Right aligned  ADC4_seq4_2_overSampling=x1 (12 bits)  ADC5_seq4_2_TXT=Not Used  ADC5_seq4_2_align=Right aligned  ADC5_seq4_2_overSampling=x1 (12 bits)  ADC1_seq4_3_TXT=Not Used  ADC1_seq4_3_align=Right aligned  ADC1_seq4_3_overSampling=x1 (12 bits)  ADC2_seq4_3_TXT=Not Used  ADC2_seq4_3_align=Right aligned  ADC2_seq4_3_overSampling=x1 (12 bits)  ADC3_seq4_3_TXT=Not Used  ADC3_seq4_3_align=Right aligned  ADC3_seq4_3_overSampling=x1 (12 bits)  ADC4_seq4_3_TXT=Not Used  ADC4_seq4_3_align=Right aligned  ADC4_seq4_3_overSampling=x1 (12 bits)  ADC5_seq4_3_TXT=Not Used  ADC5_seq4_3_align=Right aligned  ADC5_seq4_3_overSampling=x1 (12 bits)  ADC1_seq4_4_TXT=Not Used  ADC1_seq4_4_align=Right aligned  ADC1_seq4_4_overSampling=x1 (12 bits)  ADC2_seq4_4_TXT=Not Used  ADC2_seq4_4_align=Right aligned  ADC2_seq4_4_overSampling=x1 (12 bits)  ADC3_seq4_4_TXT=Not Used  ADC3_seq4_4_align=Right aligned  ADC3_seq4_4_overSampling=x1 (12 bits)  ADC4_seq4_4_TXT=Not Used  ADC4_seq4_4_align=Right aligned  ADC4_seq4_4_overSampling=x1 (12 bits)  ADC5_seq4_4_TXT=Not Used  ADC5_seq4_4_align=Right aligned  ADC5_seq4_4_overSampling=x1 (12 bits)  ADC1_seq4_5_TXT=Not Used  ADC1_seq4_5_align=Right aligned  ADC1_seq4_5_overSampling=x1 (12 bits)  ADC2_seq4_5_TXT=Not Used  ADC2_seq4_5_align=Right aligned  ADC2_seq4_5_overSampling=x1 (12 bits)  ADC3_seq4_5_TXT=Not Used  ADC3_seq4_5_align=Right aligned  ADC3_seq4_5_overSampling=x1 (12 bits)  ADC4_seq4_5_TXT=Not Used  ADC4_seq4_5_align=Right aligned  ADC4_seq4_5_overSampling=x1 (12 bits)  ADC5_seq4_5_TXT=Not Used  ADC5_seq4_5_align=Right aligned  ADC5_seq4_5_overSampling=x1 (12 bits)  ADC_TRG2_ACCBRST_seq4=Burst - not interruptible  ADC1_NINSEL_seq4_TXT=Vss - single ended (unsigned)  ADC2_NINSEL_seq4_TXT=Vss - single ended (unsigned)  ADC3_NINSEL_seq4_TXT=Vss - single ended (unsigned)  ADC4_NINSEL_seq4_TXT=Vss - single ended (unsigned)  ADC5_NINSEL_seq4_TXT=Vss - single ended (unsigned)  TrigTimeStep_seq4=on  info_seq4=0  TrigSource_seq5_TXT=PWM1 adc trig 1  SampleTime_seq5_Tad_TXT="4.5 Tad  = 56.2ns  -  Rin < 5.2 kOhm"  ADC1_seq5_TXT=AD1 AN0 / A2 / Pin[25]  ADC1_seq5_align=Left aligned  ADC1_seq5_overSampling=x1 (12 bits)  ADC2_seq5_TXT=AD2 AN0 / B0 / Pin[41]  ADC2_seq5_align=Right aligned  ADC2_seq5_overSampling=x1 (12 bits)  ADC3_seq5_TXT=Not Used  ADC3_seq5_align=Left aligned  ADC3_seq5_overSampling=x1 (12 bits)  ADC4_seq5_TXT=AD4 AN0 / B4 / Pin[57]  ADC4_seq5_align=Left aligned  ADC4_seq5_overSampling=x1 (12 bits)  ADC5_seq5_TXT=AD5 AN0 / A7 / Pin[5]  ADC5_seq5_align=Left aligned  ADC5_seq5_overSampling=x1 (12 bits)  ADC1_seq5_1_TXT=Not Used  ADC1_seq5_1_align=Right aligned  ADC1_seq5_1_overSampling=x1 (12 bits)  ADC2_seq5_1_TXT=Not Used  ADC2_seq5_1_align=Right aligned  ADC2_seq5_1_overSampling=x1 (12 bits)  ADC3_seq5_1_TXT=Not Used  ADC3_seq5_1_align=Right aligned  ADC3_seq5_1_overSampling=x1 (12 bits)  ADC4_seq5_1_TXT=Not Used  ADC4_seq5_1_align=Right aligned  ADC4_seq5_1_overSampling=x1 (12 bits)  ADC5_seq5_1_TXT=Not Used  ADC5_seq5_1_align=Right aligned  ADC5_seq5_1_overSampling=x1 (12 bits)  ADC1_seq5_2_TXT=Not Used  ADC1_seq5_2_align=Right aligned  ADC1_seq5_2_overSampling=x1 (12 bits)  ADC2_seq5_2_TXT=Not Used  ADC2_seq5_2_align=Right aligned  ADC2_seq5_2_overSampling=x1 (12 bits)  ADC3_seq5_2_TXT=Not Used  ADC3_seq5_2_align=Right aligned  ADC3_seq5_2_overSampling=x1 (12 bits)  ADC4_seq5_2_TXT=Not Used  ADC4_seq5_2_align=Right aligned  ADC4_seq5_2_overSampling=x1 (12 bits)  ADC5_seq5_2_TXT=Not Used  ADC5_seq5_2_align=Right aligned  ADC5_seq5_2_overSampling=x1 (12 bits)  ADC1_seq5_3_TXT=Not Used  ADC1_seq5_3_align=Right aligned  ADC1_seq5_3_overSampling=x1 (12 bits)  ADC2_seq5_3_TXT=Not Used  ADC2_seq5_3_align=Right aligned  ADC2_seq5_3_overSampling=x1 (12 bits)  ADC3_seq5_3_TXT=Not Used  ADC3_seq5_3_align=Right aligned  ADC3_seq5_3_overSampling=x1 (12 bits)  ADC4_seq5_3_TXT=Not Used  ADC4_seq5_3_align=Right aligned  ADC4_seq5_3_overSampling=x1 (12 bits)  ADC5_seq5_3_TXT=Not Used  ADC5_seq5_3_align=Right aligned  ADC5_seq5_3_overSampling=x1 (12 bits)  ADC1_seq5_4_TXT=Not Used  ADC1_seq5_4_align=Right aligned  ADC1_seq5_4_overSampling=x1 (12 bits)  ADC2_seq5_4_TXT=Not Used  ADC2_seq5_4_align=Right aligned  ADC2_seq5_4_overSampling=x1 (12 bits)  ADC3_seq5_4_TXT=Not Used  ADC3_seq5_4_align=Right aligned  ADC3_seq5_4_overSampling=x1 (12 bits)  ADC4_seq5_4_TXT=Not Used  ADC4_seq5_4_align=Right aligned  ADC4_seq5_4_overSampling=x1 (12 bits)  ADC5_seq5_4_TXT=Not Used  ADC5_seq5_4_align=Right aligned  ADC5_seq5_4_overSampling=x1 (12 bits)  ADC1_seq5_5_TXT=Not Used  ADC1_seq5_5_align=Right aligned  ADC1_seq5_5_overSampling=x1 (12 bits)  ADC2_seq5_5_TXT=Not Used  ADC2_seq5_5_align=Right aligned  ADC2_seq5_5_overSampling=x1 (12 bits)  ADC3_seq5_5_TXT=Not Used  ADC3_seq5_5_align=Right aligned  ADC3_seq5_5_overSampling=x1 (12 bits)  ADC4_seq5_5_TXT=Not Used  ADC4_seq5_5_align=Right aligned  ADC4_seq5_5_overSampling=x1 (12 bits)  ADC5_seq5_5_TXT=Not Used  ADC5_seq5_5_align=Right aligned  ADC5_seq5_5_overSampling=x1 (12 bits)  ADC_TRG2_ACCBRST_seq5=Burst - not interruptible  ADC1_NINSEL_seq5_TXT=Vss - single ended (unsigned)  ADC2_NINSEL_seq5_TXT=Vss - single ended (unsigned)  ADC3_NINSEL_seq5_TXT=Vss - single ended (unsigned)  ADC4_NINSEL_seq5_TXT=Vss - single ended (unsigned)  ADC5_NINSEL_seq5_TXT=Vss - single ended (unsigned)  TrigTimeStep_seq5=on  info_seq5=0
      settings: SourceProductName=MPLAB Device Blocks for Simulink
  Bitwise NOT : simulink/Logic and Bit Operations/Bitwise Operator  logicop=NOT  UseBitMask=off  BitMask=bin2dec('11011001')  BitMaskRealWorld=Stored Integer
      settings: LibrarySourceBlock=|
      | simulink/Quick Insert/Logic and Bit
      | Operations/Bitwise NOT
  Buffer : Buffer  N=5  OutputFrames=off
  Chirp : dspsrcs4/Chirp  sweep=Linear  mode=Bidirectional  f0=0.1  f1=10  t1=15  Tsweep=15  phase=0  Ts=.001  spf=1  datatype=single  OutputFrames=off
  Compiler Options : MCHP_Blockset/System Configuration/Compiler Options  Priority=1  LATEST_CMPLR=off  COMP_LIST_TXT=XC-DSC - v4.00_TC1  DFP_LIST_TXT=v 0.1.201  CMSIS_DSP_TXT=Dynamic Options  USE_64BIT_DOUBLE=on  MCHP_MULTITHREAD_COMPILATION=on  UseCustom_LinkerScript=off  MCHP_MASTERLINK=PICOOZ_OL_ExtMode_Curiosity_dsPIC33AK512MPS512/Microchip Master  OPTIMIZATION_LEVEL=2  MPLAB_LINKLIB=default  MPLAB_LINKLIB1=fast floating-point math  CodeReplacement_TXT=None  OPTIMIZATION_FLTO=off  OPTIMIZATION_REORDER=off  OPTIMIZATION_ASM_REORDER=on  UNROLL_LOOPS=off  PROCEDURAL_ABSTRACTION=off  CONSERVE_STACK=off  GC_SECTIONS=None  MCODE=is less than 32768 (faster)  MCONST=in data memory  MDATA=Can use all available memory  MSCALAR=Use only memory below address 8192 (faster)  MLARGEARRAY=off  MAGGREGATE=on  HEAP_SIZE=0  OMF=elf  DEBUG_INFO=on  MCHP_STACK_USAGE=off  GCC_STACK_USAGE=off  ProduceHexOutput=off  AssemblyListing=off  SaveTemps=off  NO_EDS_WARN=on  PRINT_STATISTICS=off
      settings: SourceProductName=MPLAB Device Blocks for Simulink
  Constant : Constant  OutDataTypeStr=single  SampleTime=.001
  Counter Limited : simulink/Sources/Counter Limited  uplimit=13  tsamp=0.05
  Dashboard Scope : DashboardScope  ShowInitialText=off  TimeSpan=5  Ymin=0  Ymax=65535  ScaleAtStop=off  UpdateMode=Scroll  TicksPosition=Inside  FontColor=[0.0, 0.0, 0.0]
  Direct Lookup Table (n-D) Chenillard : LookupNDDirect  NumberOfTableDimensions=1  Table=uint16(2.^[[8:15] [14:-1:9]] )  RemoveProtectionInput=on
  Display : Display
  Gain : Gain  Gain=320e-9/0.02*100  OutDataTypeStr=single
  Half Gauge : SemiCircularGaugeBlock  TickInterval=10  FontColor=[0.0, 0.0, 0.0]
  LED [0-8]1 : MCHP_Blockset/Digital IO/Digital Output Write  PORT_TXT="C   [ 0 : 15 ]"  PIN=[8 9 10 11 12 13 14 15]  INIT_VALUE=-1  PACK=on  OUTPUT_PIN_MODE=Push-Pull (default)  SIMULTANEOUS=off  ORDERING=None  SampleTime=-1  MCHP_PORT={Digital Out}{DOU}1:1:C8;{Digital Out}{DOU}1:1:C9;{Digital Out}{DOU}1:1:C10;{Digital Out}{DOU}1:1:C11;{Digital Out}{DOU}1:1:C12;{Digital Out}{DOU}1:1:C13;{Digital Out}{DOU}1:1:C14;{Digital Out}{DOU}1:1:C15;  MCHP_MASTERLINK=PICOOZ_OL_ExtMode_Curiosity_dsPIC33AK512MPS512/Microchip Master
      settings: SourceProductName=MPLAB Device Blocks for Simulink
  MCU Load : MCHP_Blockset/Profiling/MCU Load  MCULoadPin_TXT=None  MCULoadMeasure=on  TIMER_Resolution_TXT="Resol: 0.32(us)  -  Max: 21(ms)"  MCHP_TIMER_REQUEST={MCU_Load}{MCU_Load}21:5:0:0:[]:2097152;  MCHP_TIMER_RESULT=[4 65535 ]  MCHP_MASTERLINK=PICOOZ_OL_ExtMode_Curiosity_dsPIC33AK512MPS512/Microchip Master  MCHP_COMPILED_INFO="CompiledSampleTime= [0.020000000000000000416   0 ];CompiledInportDataTypes=[    ];CompiledInportDataWidth=[];"  Info="Timer 4:  Resol: 320(ns)  -  Max: 20.9715(ms)"  SampleTime=0.02
      settings: SourceProductName=MPLAB Device Blocks for Simulink
  MCU load in % : Display
  Manual Switch : ManualSwitch
  Manual Switch1 : ManualSwitch  CurrentSetting=0
  Median : dspstat3/Median  sortAlg=Quick sort  directionMode=Entire input  dimension=1  roundingMode=Floor  overflowMode=off  accumDataTypeStr=Inherit: Same as product output  accumLastDataTypeStr=Inherit: Same as product output  outputDataTypeStr=Inherit: Same as accumulator  outputMin=[]  outputMax=[]  outputLastDataTypeStr=Inherit: Same as accumulator
      settings: allowOverrides=off
  Microchip Master : MCHP_Blockset/System Configuration/Microchip Master  Priority=1  PICREF=33AK512MPS512  TIMESTEP_REF=PWM3_Trg1 + ADC  BUSYFLAG=Dynamic Options  BUSYFLAG_TXT=None  VDD_range=Dynamic Options  PWRTEN=Not used  BOREN=Enabled  BODENV=2.7V  BORV=Not used  FPWRT=128ms  DSBOREN=Disable ZPBOR during Deep Sleep Mode  DSLPBOR=Not used  MCLRE=Enabled  SMCLR=MCLR pin generates a normal system Reset  PMDL1WAY=Allow only one reconfiguration  RSTPRI=Device will obtain reset instruction from Primary flash  TEMP=Not used  SOSCSRC=Not used  SOSCSEL=Not used  IOL1WAY=Allow only one reconfiguration  ALTVREF=Not used  DISUVREG=Not used  DSSWEN=Not used  LPCFG=Not used  RTCBAT=Not used  VBTBOR=Not used  WUTSEL=Not used  POWERSAVE=off  FNOSC=Internal Fast RC (FRC)  FPR=ECIO w/ PLL 16x  FOSFPR=HS3 w/PLL 16x  FOS=Primary Oscillator  FRANGE=High Range  OSCILLATOR_SELECT=External Clock  OSCILLATOR_SELECT_spd=External Clock  QUARTZ=8e6  QUARTZ_spd=8e6  POSCGAIN=2x gain setting  POSCBOOST=Boost the kick start of the oscillator  SOSCGAIN=2x gain setting  SOSCBOOST=Boost the kick start of the oscillator  ACTIV_PLL=on  ACTIV_PLL_spd=on  MIPS_DESIRED=200e6  MIPS_DESIRED_spd=200e6  CPUDIV=Divide by 1  FPLLMUL=Not used  FPLLIDIV=8x Divider  POSCFREQ=Not used  POSCMD=Primary Oscillator Disabled  POSCMOD=Primary osc disabled  MIPS=200 * 1e6  ACLKCON=Optimized for PWM resolution & ADC conversion speed  ACLKCON_spd=Optimized for PWM resolution & ADC conversion speed  FPLLODIV=32x Divider  PLLKEN=Clock switch to PLL source will wait until the PLL lock signal is valid  FCKSM=Both Clock switching and Fail-safe Clock Monitor are disabled  FCKSMEN=Sw Disabled; Mon Disabled  IESO=Start up with FRC; then switch  DSWDTPS=1:2^36  FWDTEN=Disable  FWDTWINSZ=Window size is 25%  FWPSA=1:512  FWPSA0=1:128  FWPSB=1:16  WDT=Disable  WDTPOST=1:32768  WDTPRE=1:128  WDTPS=1:1048576  WINDIS=Watchdog Timer in Non-Window mode  WWDTEN=Window mode  DSWDTEN=Disable DSWDT during Deep Sleep Mode  DSWDTOSC=Select LPRC as DSWDT Reference clock  FWDT_RCLKSEL=WDT Run Mode uses BFRC:256  FWDT_RWDTPS=1:2147483648  FWDT_SWDTMPS=1:2147483648  FWDT_WDTEN=Enable  FWDT_WDTRSTEN=WDT event generates a reset  FWDT_WDTWIN=WDT Window is 25% of WDT period  FWDT_WINEN=Not used  FPBDIV=Not used  FSOSCEN=Disable Secondary Oscillator  LPRCSEL=Not used  OSCIOFCN=Not used  OSCIOFNC=general purpose digital I/O pin  LVRCFG=Not used  PLL_96MHZ=Not used  PLL96MHZ=Not used  PLLDIV=Not used  WDTCLK=Not used  WDTCMX=Not used  WDTWIN=Watchdog Window is 25% of WDT period  XTCFG=24-32 MHz crystals  XTBST=Boost the kick-start  APL=Aux Flash Code protect is disabled  APLK=Aux Flash Write Protection or Code Protection is Enabled  AWRP=Auxiliary program memory is not write-protected  BSS=No Boot program Flash segment  BWP=Not used  BWRP=Boot Segment may be written  CP=Protection Disabled  EBS=No Boot EEPROM  ESS=No Segment Data EEPROM  GCP=General Segment Code protect is Disabled  GSS=General Segment Code protect is Disabled  GSS0=Not used  GSSK=General Segment Write Protection or Code Protection is Enabled  GWRP=General Segment may be written  PWP=Not used  RBS=No Boot RAM  RSS=No Secure RAM  SSS=No Secure Segment  SWRP=Secure segment may be written  WPCFG=Not used  WPDIS=Not used  WPEND=Not used  WPFP=Not used  ICESEL=Communicate on PGEC1/PGED1  ICS=Communicate on PGEC1 and PGED1  JTAGEN=Disable  FICD_JTAGEN=Disable  COE=Not used  RES=Not used  DEBUG=Debugger is disabled  BACKBUG=Not used  BKBUG=Not used  ALTI2C=I2C mapped to SDA1/SCL1 pins  ALTI2C1=SDA1/SCK1 pins are selected as the I/O pins for I2C1  ALTI2C2=SDA2/SCK2 pins are selected as the I/O pins for I2C2  ALTI2C3=I2C3 mapped to SDA3/SCL3 pins  FDEVOPT1_ALTI2C1=Not used  FDEVOPT1_ALTI2C2=Not used  FDEVOPT1_SPI2MAPDIS=Not used  FDEVOPT_ALTI2C1=Primary I2C1 pins are used  FDEVOPT_ALTI2C2=Primary I2C2 pins are used  FDEVOPT_ALTI2C3=Primary I2C3 pins are used  FDEVOPT_SPI2PIN=SPI2 pins are selected by peripheral pin selection feature  ALTQIO=QEA1; QEB1; INDX1 are selected as inputs to QEI1  ALTSS1=SS1A is selected as the I/O pin for SPI1  CMPPOL0=Hysteresis is applied to falling edge  CMPPOL1=Hysteresis is applied to falling edge  FCANIO=Not used  FETHIO=Default Ethernet I/O  FMIIEN=MII Enabled  FSRSSEL=Not used  FUSBIDIO=Controlled by the USB Module  FVBUSONIO=Not used  HPOL=PWM module high side output pins have active-high output polarity  HYST0=45 mV Hysteresis  HYST1=45 mV Hysteresis  I2C1SEL=Not used  LPOL=PWM module low side output pins have active-high output polarity  PWMPIN=PWM module pins controlled by PORT register at device Reset  RTCOSC=Not used  UPLLEN=USB PLL Disabled  UPLLIDIV=Not used  ATMOD8=Not used  ALTPMP=Not used  I2C2SEL=Not used  ALTADREF=Not used  ALTCVREF=Not used  PWMLOCK=PWM registers may be written without key sequence  INT_PRIORITY_DMA=0  MCHP_TIMER_RESULT=[ ]  MCHP_PLLRegisters="[0        -1     16386        -1  16815713]"  MCHPVAR=MCHP.fcy.MIPS=2e+08;MCHP.fcy.SYSCLK=2e+08;MCHP.fcy.Fplli=8000000;MCHP.fcy.Fvco=1.2e+09;MCHP.fcy.Fpllo=2e+08;MCHP.fcy.PWM=2e+08;MCHP.fcy.ADC=80000000;MCHP.fcy.PDM_DAC=2e+08;MCHP.fcy.UART=2e+08;MCHP.fcy.SPI=2e+08;MCHP.fcy.BiSS=2e+08;MCHP.fcy.SCC=2e+08;MCHP.fcy.Timers=1e+08;MCHP.fcy.I2C=2e+08;MCHP.PowerSave=0;MCHP.TimeStepFactor=-1000;MCHP.TimeStep_Timer=-1;MCHP.NTIMERS=3;MCHP.id.name='33AK512MPS512';MCHP.id.N=reshape([33 512 512],1,3);MCHP.id.L=reshape({ 'AK','MPS',''},1,3);MCHP.id.Arch=8;MCHP.id.maskset='STX32_Pegasus';MCHP.id.masksetFamily='STX32_Pegasus';MCHP.id.dos='05308';MCHP.id.ds='0';MCHP.id.archTxt='33Axxx';MCHP.id.clonedfrom='DSPIC33AK128MC106';MCHP.id.isSlave=0;MCHP.id.isMaster=0;MCHP.periph.PPS.reg_RPINRx=reshape([-1 1 1 1 1 1 1 1 1 1 1 1 1 1 1 1 1 1 1 1 1 1 1 1 1 1 -1 -1 -1 -1 -1 -1 1 1 1 1 1 1 1 1 1 1 1 1 1 1 1 1 1 1 1 1 1 1 1 1 1 1 1 1 1 1 1 1 1 1 1 1 1 1 1 1 1 1 1 1 1 1 1 1 1 1 1 -1 -1 -1 -1 -1 -1 -1 -1 -1 -1 1 1 1 1 1 1 1 1 1 1 1 1 1 1 1 1 1 1],1,111);MCHP.periph.pin.ODCx=reshape([65535 65535 65535 65535 2047 4079 1015 7 0 0 0],1,11);MCHP.PPS.dsPIC.RP=reshape([-1 0 1 2 3 4 5 6 7 8 9 10 11 12 13 14 15 16 17 18 19 20 21 22 23 24 25 26 27 28 29 30 31 32 33 34 35 36 37 38 39 40 41 42 43 44 45 46 47 48 49 50 51 52 53 54 55 56 57 58 59 60 61 62 63 64 65 66 67 68 69 70 71 72 73 74 -1 -1 -1 -1 -1 80 81 82 83 -1 85 86 87 88 89 90 91 -1 -1 -1 -1 96 97 98 -1 100 101 102 103 104 105 -1 -1 -1 -1 -1 -1 112 113 114],1,116);MCHP.PPS.dsPIC.RPI=[];MCHP.PPS.dsPIC.RPINR_list=reshape({ '1','INT1','INT2','INT3','INT4','T1CK','T2CK','T3CK','TCKI1','ICM1','TCKI2','ICM2','TCKI3','ICM3','TCKI4','ICM4','TCKI5','ICM5','TCKI6','ICM6','TCKI7','ICM7','TCKI8','ICM8','TCKI9','ICM9','27','28','OCFA','OCFB','OCFC','OCFD','PCI8','PCI9','PCI10','PCI11','QEIA1','QEIB1','QEINDX1','QEIHOM1','QEIA2','QEIB2','QEINDX2','QEIHOM2','QEIA3','QEIB3','QEINDX3','QEIHOM3','QEIA4','QEIB4','QEINDX4','QEIHOM4','U1RX','U1DSR','U2RX','U2DSR','U3RX','U3DSR','SDI1','SCK1_in','SS1_in','SDI2','SCK2_in','SS2_in','SDI3','SCK3_in','SS3_in','SDI4','SCK4_in','SS4_in','C1RX','C2RX','SENT1','SENT2','REFI1','REFI2','PCI12','PCI13','PCI14','PCI15','PCI16','PCI17','PCI18','CLCINA','CLCINB','CLCINC','CLCIND','CLCINE','CLCINF','CLCING','CLCINH','CLCINI','CLCINJ','ADTRG31','U1CTS','U2CTS','U3CTS','BISSSL1','BISSGS1','IOMON1F12','IOMON1F13','IOMON1F14','IOMON1F15','IOMON2F12','IOMON2F13','IOMON2F14','IOMON2F15','PCI19','PCI20','PCI21','PCI22'},1,111);MCHP.PPS.dsPIC.RPOR_list=reshape({ '1','PWM1H','PWM1L','PWM2H','PWM2L','PWM3H','PWM3L','PWM4H','PWM4L','PWM5H','PWM5L','PWM6H','PWM6L','PWM7H','PWM7L','PWM8H','PWM8L','CAN1TX','CAN2TX','U1TX','U1RTS','U2TX','U2RTS','U3TX','U3RTS','SDO1','SCK1_out','SS1_out','SDO2','SCK2_out','SS2_out','SDO3','SCK3_out','SS3_out','SDO4','SCK4_out','SS4_out','REFO1','REFO2','OCM1','OCM2','OCM3','OCM4','OCM5','OCM6','OCM7','OCM8','MCCP_OCM1A','MCCP_OCM1B','MCCP_OCM1C','MCCP_OCM1D','MCCP_OCM1E','MCCP_OCM1F','CMPO1','CMPO2','CMPO3','CMPO4','CMPO5','CMPO6','CMPO7','CMPO8','PWME1','PWME2','PWME3','PWME4','QEICMP1','QEICMP2','QEICMP3','QEICMP4','CLC1OUT','CLC2OUT','CLC3OUT','CLC4OUT','CLC5OUT','CLC6OUT','CLC7OUT','CLC8OUT','CLC9OUT','CLC10OUT','PTGTRG24','PTGTRG25','SENT1OUT','SENT2OUT','BISSMO1','BISSMA1','U1DTR','U2DTR','U3DTR','APWM1H','APWM1L','APWM2H','APWM2L','APWM3H','APWM3L','APWM4H','APWM4L','APWME1','APWME2'},1,98);MCHP.PPS.dsPIC.RPV=reshape([-1 -1 -1 -1 -1 -1],1,6);MCHP.PPS.map_RPnR_RPORx=reshape([1 2 3 4 5 6 7 8 9 10 11 12 13 14 15 16 17 18 19 20 21 22 23 24 25 26 27 28 29 30 31 32 33 34 35 36 37 38 39 40 41 42 43 44 45 46 47 48 49 50 51 52 53 54 55 56 57 58 59 60 61 62 63 64 65 66 67 68 69 70 71 72 73 74 75 -1 -1 -1 -1 -1 81 82 83 84 -1 86 87 88 89 90 91 92 -1 -1 -1 -1 97 98 99 -1 101 102 103 104 105 106 107 -1 -1 -1 -1 -1 113 114 115 -1 -1 -1 -1 -1 -1 -1 -1 -1 -1 -1 -1 -1 129 130 131 132 133 134 135 136 137 138 139 140 141 142 143 144],1,144);MCHP.Rx=reshape([4 41 79 101 1 48 65 97 -1 -1 -1 7 43 80 102 2 49 66 100 -1 -1 -1 25 44 82 106 11 50 67 103 -1 -1 -1 27 55 84 107 6 63 -1 -1 -1 -1 -1 28 57 85 117 19 -1 90 -1 -1 -1 -1 29 33 83 115 26 59 74 -1 -1 -1 -1 31 58 73 116 23 56 76 -1 -1 -1 -1 5 60 75 124 17 53 81 -1 -1 -1 -1 14 45 71 125 15 39 86 -1 -1 -1 -1 16 46 72 98 8 36 89 -1 -1 -1 -1 18 61 87 99 30 34 -1 -1 -1 -1 -1 13 62 88 118 -1 42 -1 -1 -1 -1 -1 3 35 91 119 -1 -1 -1 -1 -1 -1 -1 12 40 92 121 -1 -1 -1 -1 -1 -1 -1 24 54 95 122 -1 -1 -1 -1 -1 -1 -1 20 47 96 123 -1 -1 -1 -1 -1 -1 -1],11,16);MCHP.ADC.ANtype=reshape([3 1],1,2);MCHP.ADC.ADCONx=reshape([4294804960 0 0 0 0 0],1,6);MCHP.ADC.ADCHS_0=reshape([0 0],1,2);MCHP.ADC.Flags=reshape([1 0],1,2);MCHP.ADC.Buffer=reshape([-1 -1],1,2);MCHP.ADC.port=reshape([-1 -1 -1 -1 -1 -1 -1 -1 -1 -1 -1 -1 -1 -1 -1 -1 -1 -1 -1 -1 -1 -1 -1 -1 -1 -1 -1 -1 -1 -1 -1 -1 -1 -1 -1 -1 -1 -1 -1 -1 -1 -1 -1 -1 -1 -1 -1 -1 -1 -1 -1 -1 -1 -1 -1 -1 -1],1,57);MCHP.ADC.port_ALT=reshape([-1 -1 -1 -1],1,4);MCHP.ADC.port_ALTA=reshape([-1 -1 -1 -1],1,4);MCHP.ADC.port_ALTB=reshape([-1 -1 -1 -1],1,4);MCHP.ADC.port_ALTC=reshape([-1 -1 -1 -1],1,4);MCHP.ADC.port_VrefP=-1;MCHP.ADC.port_VrefM=-1;MCHP.ADC.port_AVdd=-1;MCHP.ADC.port_AVss=-1;MCHP.ADC.ADCDATA=reshape([0 0 0 0 0 0 0 0 0 0 0 0 0 0 0 0 0 0 0 0 0 0 0 0 0 0 0 0 0 0 0 0 0 0 0 0 0 0 0 0 0 0 0 0 0 0 0 0 0 0 0 0 0 0 0 0 0],1,57);MCHP.ADC.HS_SAR.TRGSRC=reshape([0 0 0 0 0 0 0 0 0 0 0 0 0 0 0 0 0 0 0 0 0 0 0 0 0 0 0 0 0 0 0 0],1,32);MCHP.ADC.HS_SAR.nFilters=0;MCHP.ADC.HS_SAR.nDedicatedCore=0;MCHP.ADC.HS_SAR.CALIBRATION=0;MCHP.ADC.HS_SAR.ADCON1L=-1;MCHP.ADC.HS_SAR.ADC_Class3_idxStart=32;MCHP.memory.RAM=32768;MCHP.memory.RAM_XBegin=16384;MCHP.memory.RAM_YBegin=49152;MCHP.memory.RAM_dma=reshape([-1 -1],1,2);MCHP.memory.FLASH_ECC=0;MCHP.DMA.Num=8;MCHP.DMA.CNTmax=16777215;MCHP.QEI.QEICONx=reshape([49023 49023 49023 49023 -1 -1],1,6);MCHP.QEI.QEItype=4;MCHP.QEI.Port_QEI_INDX=reshape([-1 -1],1,2);MCHP.QEI.Port_QEI_QEA=reshape([-1 -1],1,2);MCHP.QEI.Port_QEI_QEB=reshape([-1 -1],1,2);MCHP.QEI.Port_QEI_UPDN=reshape([-1 -1],1,2);MCHP.INT.Port=reshape([5 32767 32767 32767 32767],1,5);MCHP.ADC1.port=reshape([2 4 3 9 10 -1 -1 -1 -1 -1 -1 -1 -1 -1 -1 -1 -1 -1 -1 -1 -1 -1 -1 -1 -1 -1 -1 -1 -1 -1 -1 -1],1,32);MCHP.ADC2.port=reshape([16 18 17 25 24 31 -1 -1 -1 -1 -1 -1 -1 -1 -1 -1 -1 -1 -1 -1 -1 -1 -1 -1 -1 -1 -1 -1 -1 -1 -1 -1],1,32);MCHP.ADC3.port=reshape([5 21 6 29 80 0 -1 -1 -1 -1 -1 -1 -1 -1 -1 -1],1,16);MCHP.ADC4.port=reshape([20 22 23 19 26 21 -1 -1 -1 -1 -1 -1 -1 -1 -1 -1],1,16);MCHP.ADC5.port=reshape([7 1 11 8 4 -1 -1 -1 -1 -1 -1 -1 -1 -1 -1 -1],1,16);MCHP.ADC1N.port=reshape([-1 10 3 -1 -1 -1 -1 -1 -1 -1],1,10);MCHP.ADC2N.port=reshape([-1 25 17 -1 -1 -1 -1 -1 -1 -1],1,10);MCHP.ADC3N.port=reshape([-1 29 6 -1],1,4);MCHP.ADC4N.port=reshape([-1 23 22 -1],1,4);MCHP.ADC5N.port=reshape([-1 7 11 -1],1,4);MCHP.PWM_HS.Flags=reshape([0 0 0],1,3);MCHP.PWM.port_FLT=reshape([-1 -1 -1 -1 -1 -1 -1 -1 -1 -1 -1 -1 -1 -1 -1 -1 -1 -1 -1 -1 -1 -1 -1 -1 -1 -1 -1 -1 -1 -1 -1 -1 -1],1,33);MCHP.PWM.PWMRef=-1;MCHP.PWM.Flag=0;MCHP.PWM.Port_PWM_l=reshape([51 40 49 63 36 47 37 98 54 -1 58 -1 43 -1 45 -1 -1 -1 -1 -1 -1 -1 -1 -1],2,12);MCHP.PWM.Port_PWM_h=reshape([50 59 48 62 35 46 34 97 53 -1 57 -1 42 -1 44 -1 -1 -1 -1 -1 -1 -1 -1 -1],2,12);MCHP.PWM_HS_FEP.nEVTOUT=5;MCHP.IC.Port=reshape([0 0 0 0 0 0 0 0 0 0 0 0 0 0 0 0],1,16);MCHP.IC.type=-1;MCHP.OC.Port=reshape([0 0 0 0 0 0 0 0 0 0 0 0 0 0 0 0],1,16);MCHP.OC.type=-1;MCHP.CN.Port=reshape([-1 -1 -1 -1 -1 -1 -1 -1 -1 -1 -1 -1 -1 -1 -1 -1 -1 -1 -1 -1 -1 -1 -1 -1 -1 -1 -1 -1 -1 -1 -1 -1 -1 -1 -1 -1 -1 -1 -1 -1 -1 -1 -1 -1 -1 -1 -1 -1 -1 -1 -1 -1 -1 -1 -1 -1 -1 -1 -1 -1 -1 -1 -1 -1 -1 -1 -1 -1 -1 -1 -1 -1 -1 -1 -1 -1 -1 -1 -1 -1 -1 -1 -1 -1 -1],1,85);MCHP.CN.PullUp=reshape([65535 65535 65535 65535 2047 4079 1015 7 0 0 0],1,11);MCHP.CN.type=2;MCHP.CN.Flag_PullDown=1;MCHP.SPI.Refs=reshape([1 2 3 4 0 0],1,6);MCHP.SPI.SPIxCON1=-1;MCHP.SPI.SPIxCON2=-1;MCHP.SPI.SPIxFIFOSIZE=4;MCHP.SPI.Port_SDI=reshape([-1 27 -1 -1 -1 -1],1,6);MCHP.SPI.Port_SDO=reshape([-1 41 -1 -1 -1 -1],1,6);MCHP.SPI.Port_SCK=reshape([-1 26 -1 -1 -1 -1],1,6);MCHP.SPI.Port_SS=reshape([-1 -1 -1 -1 -1 -1],1,6);MCHP.I2C.Refs=reshape([1 2 3 0 0],1,5);MCHP.I2C.I2CxCON=58703615;MCHP.I2C.NewRegName=4;MCHP.I2C.Port_SDA=reshape([19 7 39 -1 -1],1,5);MCHP.I2C.Port_SCL=reshape([20 0 38 -1 -1],1,5);MCHP.I2C.Port_ASDA=reshape([54 56 60 -1 -1],1,5);MCHP.I2C.Port_ASCL=reshape([53 55 52 -1 -1],1,5);MCHP.I2C.Fuse_Port_SCL_SDA=reshape([7 1 8 1 9 1 -1 -1 -1 -1],2,5);MCHP.I2C.Fuse_Port_ASCL_ASDA=reshape([7 2 8 2 9 2 -1 -1 -1 -1],2,5);MCHP.SCCP.nSCCP=9;MCHP.SCCP.MCCP=reshape([1 1 1 1 1 1 1 1 1],1,9);MCHP.PGA.Port_PGA1P=reshape([-1 -1 -1 -1],1,4);MCHP.PGA.Port_PGA1N=reshape([-1 -1 -1 -1],1,4);MCHP.PGA.Port_PGA2P=reshape([-1 -1 -1 -1],1,4);MCHP.PGA.Port_PGA2N=reshape([-1 -1 -1 -1],1,4);MCHP.PGA.Num=0;MCHP.HS_AnalogComparator.Port_CMP1=reshape([2 4 3 14],1,4);MCHP.HS_AnalogComparator.Port_CMP2=reshape([16 18 17 24],1,4);MCHP.HS_AnalogComparator.Port_CMP3=reshape([5 21 6 28],1,4);MCHP.HS_AnalogComparator.Port_CMP4=reshape([19 20 23 1],1,4);MCHP.HS_AnalogComparator.Port_CMP5=reshape([8 9 10 13],1,4);MCHP.HS_AnalogComparator.Port_CMP6=reshape([0 7 11 -1],1,4);MCHP.HS_AnalogComparator.Port_CMP7=reshape([9 27 64 22],1,4);MCHP.HS_AnalogComparator.Port_CMP8=reshape([26 30 65 25],1,4);MCHP.HS_AnalogComparator.Port_CMPN=reshape([-1 -1 3 6 10 11],1,6);MCHP.HS_AnalogComparator.Port_EXTREFx=reshape([-1 -1],1,2);MCHP.HS_AnalogComparator.Port_DACOUTx=reshape([1 8],1,2);MCHP.HS_AnalogComparator.Num=8;MCHP.Comp.Port_CVrefin=-1;MCHP.Comp.Port_CVref=-1;MCHP.Comp.Port_CVref1O=-1;MCHP.Comp.Port_CVref2O=-1;MCHP.Comp.Port_CxOUT=reshape([32767 32767 32767 32767 32767],1,5);MCHP.Comp.Port_OAxOUT=reshape([2 16 5 -1 -1],1,5);MCHP.Comp.Port_CxINP=reshape([-1 -1 -1 -1 -1],1,5);MCHP.Comp.Port_CxINM=reshape([-1 -1 -1 -1 -1 -1 -1 -1 -1 -1 -1 -1 -1 -1 -1 -1 -1 -1 -1 -1],4,5);MCHP.Comp.Port_OAxINP=reshape([4 18 21 -1 -1],1,5);MCHP.Comp.Port_OAxINM=reshape([3 17 6 -1 -1],1,5);MCHP.Comp.nComp=reshape([5 0 0],1,3);MCHP.Comp.OpAmp=0;MCHP.Comp.CVRCON=reshape([0 0],1,2);MCHP.Comp.CMCON=0;MCHP.CDAC.Port_DACx=reshape([-1 -1 -1],1,3);MCHP.CDAC.nCDAC=8;MCHP.UART.port_Rx=reshape([32767 32767 32767 -1 -1 -1],1,6);MCHP.UART.port_Tx=reshape([32767 32767 32767 -1 -1 -1],1,6);MCHP.UART.port_ARx=reshape([-1 -1],1,2);MCHP.UART.port_ATx=reshape([-1 -1],1,2);MCHP.UART.port_RTS=reshape([32767 32767 32767 -1 -1 -1],1,6);MCHP.UART.port_CTS=reshape([32767 32767 32767 -1 -1 -1],1,6);MCHP.UART.reg_UxMODE=reshape(MCHP_Fun.Hex2num('[41E9FFF77FE00000 41E9FFF77FE00000 41E9FFF77FE00000 BFF0000000000000 BFF0000000000000 BFF0000000000000]'),1,6);MCHP.UART.reg_UxSTA=reshape(MCHP_Fun.Hex2num('[41DDFFFFFFC00000 41DDFFFFFFC00000 41DDFFFFFFC00000 BFF0000000000000 BFF0000000000000 BFF0000000000000]'),1,6);MCHP.modsrc.DOS_04094_cpu_33a_v1_dspic33a=1;MCHP.modsrc.DOS_04436_perseus_dspic33a=0;MCHP.modsrc.DOS_04928_gpio_ports_upb_v2_dspic33a=1;MCHP.modsrc.DOS_02672_math_progcrc_upb_v1_dspic33a=1;MCHP.modsrc.DOS_04993_sec_32bit_cp_upb_v1_dspic33a=1;MCHP.modsrc.DOS_03459_adc_pc_ctrl_upb_v2_dspic33a=0;MCHP.modsrc.DOS_04302_pwm_pc_upb_v3_dspic33a=0;MCHP.modsrc.DOS_03076_uart_protocol_upb_v1_dspic33a=1;MCHP.modsrc.DOS_01482_spi_i2s_upb_v1_dspic33a=1;MCHP.modsrc.DOS_05155_i2c_upb_v4_dspic33a=1;MCHP.modsrc.DOS_02359_sent_j2716_upb_v1_dspic33a=1;MCHP.modsrc.DOS_05177_qei_32b_upb_v2_dspic33a=1;MCHP.modsrc.DOS_01512_ccp_mccp_upb_v1_dspic33a=1;MCHP.modsrc.DOS_03496_dac_pdm_nbit_upb_v2_dspic33a=0;MCHP.modsrc.DOS_02673_tmr_classa_upb_v1_dspic33a=1;MCHP.modsrc.DOS_04776_perf_mon_upb_v1_dspic33a=1;MCHP.modsrc.DOS_03680_pfm_pbu_33a_upb_v1_dspic33a=1;MCHP.modsrc.DOS_04649_sec_pac_upb_v0_dspic33a=0;MCHP.modsrc.DOS_03966_io_integrity_monitor_upb_v1_dspic33a=1;MCHP.modsrc.DOS_04641_biss_master_upb_v1_dspic33a=1;MCHP.modsrc.DOS_04077_dma_upb_v1_dspic33a=1;MCHP.modsrc.DOS_04549_nvm_ctrl_32bit_upb_v1_dspic33a=1;MCHP.modsrc.DOS_04449_clk_cru_33a_upb_v1_dspic33a=1;MCHP.modsrc.DOS_03850_clk_monitor_upb_v1_dspic33a=1;MCHP.modsrc.DOS_04342_osc_rc8mhz_ctrl_upb_v4_dspic33a=1;MCHP.modsrc.DOS_04650_wdt_upb_v4_dspic33a=1;MCHP.modsrc.DOS_05178_ptg_pc_upb_v2_dspic33a=1;MCHP.modsrc.DOS_04181_data_ram_ctrl_upb_v1_dspic33a=1;MCHP.modsrc.DOS_04735_wdt_dmt_upb_v6_dspic33a=1;MCHP.modsrc.DOS_01577_cla_clc_upb_v1_dspic33a=1;MCHP.modsrc.DOS_03516_pwr_sib_upb_v3_dspic33a=0;MCHP.modsrc.DOS_03495_amp_pad_opamp_ctrl_upb_v2_dspic33a=1;MCHP.modsrc.DOS_05830_blueRidge_dspic33a=0;MCHP.modsrc.DOS_05972_adc_12b_upb_v3_itc_dspic33a=0;MCHP.modsrc.DOS_05404_adc_pc_ctrl_upb_v3_dspic33a=1;MCHP.modsrc.DOS_05226_pwm_pc_upb_v4_dspic33a=1;MCHP.modsrc.DOS_05514_qei_32b_upb_v3_dspic33a=0;MCHP.modsrc.DOS_05431_dac_pdm_nbit_upb_v3_dspic33a=1;MCHP.modsrc.DOS_05828_pfm_pbu_33a_upb_v2_dspic33a=0;MCHP.modsrc.DOS_05765_math_rdc_upb_v1_32bit=0;MCHP.modsrc.DOS_05908_math_cic_upb_v2_32bit=0;MCHP.modsrc.DOS_05801_dma_upb_v2_dspic33a=0;MCHP.modsrc.DOS_05461_pwr_sib_upb_v4_dspic33a=1;MCHP.modsrc.DOS_05420_amp_vref_ctl_upb_v1_dspic33a=1;MCHP.modsrc.DOS_05592_pwr_monitor_sib_upb_v1=0;MCHP.modsrc.DOS_05924_bus_dual_die_upb_v2=0;MCHP.modsrc.DOS_06048_sec_cam_v3_dspic33a=0;MCHP.modsrc.DOS_05922_i3c_upb_v1_32bit=0;MCHP.modsrc.DOS_06006_adc_soft_code_seq_v2_dspic33a=0;MCHP.modsrc.DOS_05442_icd_trace_33a_v1_dspic33a=0;MCHP.modsrc.DOS_04537_can_fd_upb_v3_dspic33a=1;MCHP.modsrc.DOS_05308_pegasus_dspic33a=1;MCHP.modsrc.DOS_02976_adc_12b_upb_v2_dspic33a=1;MCHP.modsrc.DOS_05226_apwm_pc_upb_v4_dspic33a=1;MCHP.modsrc.DOS_04649_sec_pac_upb_v1_dspic33a=1;MCHP.modsrc.DOS_05346_sec_cam_v2_dspic33a=1;MCHP.modsrc.DOS_03267_adc_soft_code_seq_v1_dspic33a=1;MCHP.modsrc.DOS_05557_serpens_dspic33a=0;MCHP.modsrc.DOS_05972_adc_12b_upb_v3_adc_dspic33a=0;MCHP.modsrc.DOS_03681_bmx_33a_upb_v1_dspic33a=0;MCHP.modsrc.DOS_02050_tmr_rtcc_upb_v1_dspic33a=0;MCHP.modsrc.DOS_04649_sec_pac_upb_serpens_dspic33a=0;MCHP.modsrc.DOS_05692_pwr_sib_upb_v5_dspic33a=0;MCHP.modsrc.DOS_06006_adc_soft_code_seq_v2_adc_dspic33a=0;MCHP.modsrc.DOS_02551_cpu_16bit_v7=0;MCHP.modsrc.DOS_01520_wdt_dmt_upb_v1_16bit=0;MCHP.modsrc.DOS_02359a_sent_j2716_upb_v1=0;MCHP.modsrc.DOS_02672_math_progcrc_upb_v1_16bit=0;MCHP.modsrc.DOS_01577_cla_clc_upb_v1=0;MCHP.modsrc.DOS_02915_ecc_v2=0;MCHP.modsrc.DOS_02673_tmr_classa_upb_v1_16bit=0;MCHP.modsrc.DOS_01494_qei_32b_upb_v1_16bit=0;MCHP.modsrc.DOS_02472_ppi_pmp16_upb_v1_16bit=0;MCHP.modsrc.DOS_01441_i2c_upb_v1_16bit_TLAH=0;MCHP.modsrc.DOS_03076_uart_protocol_upb_v1_16bit=0;MCHP.modsrc.DOS_01482=0;MCHP.modsrc.DOS_01483_pwm_16bit=0;MCHP.modsrc.DOS_02949_WACG=0;MCHP.modsrc.DOS_02316_nvm_ctrl_v1_16bit=0;MCHP.modsrc.DOS_03349_amp_pad_opamp_ctrl_upb_v1=0;MCHP.modsrc.DOS_02653_afe_current_bias_ctrl_upb_v1_16bit=0;MCHP.modsrc.DOS_01459_ptg_pc_upb_v1_16bit=0;MCHP.modsrc.DOS_01512_ccp_mccp_upb_v1_16bit=0;MCHP.modsrc.DOS_02519_dma_sfr_16bit_v2=0;MCHP.modsrc.DOS_02508c11=0;MCHP.modsrc.DOS_02475_dac_pdm_nbit_upb_v1_16bit=0;MCHP.modsrc.DOS_02467_gpio_upb_v1_16bit=0;MCHP.modsrc.DOS_00805_rst_integration_v4=0;MCHP.modsrc.DOS_02659_clk_sib_v12=0;MCHP.modsrc.DOS_02237_osc_dco_ctrl_upb_v1_16bit=0;MCHP.modsrc.DOS_02674_wdt_upb_v1_16bit=0;MCHP.modsrc.DOS_01407=0;MCHP.modsrc.DOS_03247_CAN_FD_UPB_V2_16_bit=0;MCHP.modsrc.DOS_03994_WAC07=0;MCHP.modsrc.DOS_02552_msi_upb_v1_Master=0;MCHP.modsrc.DOS_03667_pwm_pc_upb_v2_16bit=0;MCHP.modsrc.DOS_04180_drm_ctrl_ecc_v1=0;MCHP.modsrc.DOS_03431_STX03=0;MCHP.modsrc.DOS_03516_pwr_sib_upb_v3=0;MCHP.modsrc.DOS_02552_msi_upb_v1_Slave=0;MCHP.modsrc.DOS_04621_amp_pga_ctrl_upb_v3=0;MCHP.modsrc.DOS_02497_WACV=0;MCHP.modsrc.DOS_02593_amp_pga_ctrl_pb_v2_16bit=0;MCHP.modsrc.DOS_01461_afe_ctmu_con_upb_v1_16bit=0;MCHP.modsrc.DOS_02497_WACA=0;MCHP.modsrc.DOS_02478_uart_irda_upb_v1_16bit=0;MCHP.modsrc.DOS_00929=0;MCHP.modsrc.DOS_01198=0;MCHP.modsrc.DOS_03029_WACH=0;MCHP.modsrc.DOS_01483_apwm_16bit=0;MCHP.modsrc.DOS_04797_WAC0A=0;MCHP.modsrc.DOS_04884_WAC0B=0;MCHP.modsrc.DOS_04797_WAC09=0;MCHP.modsrc.DOS_03662_WACU=0;MCHP.modsrc.DOS_00794=0;MCHP.modsrc.DOS_00931=0;MCHP.modsrc.DOS_00932=0;MCHP.modsrc.DOS_00942=0;MCHP.modsrc.DOS_00938=0;MCHP.modsrc.DOS_00996=0;MCHP.modsrc.DOS_00997=0;MCHP.modsrc.DOS_00998=0;MCHP.modsrc.DOS_00209=0;MCHP.modsrc.DOS_01555_adc=0;MCHP.modsrc.DOS_01293=0;MCHP.modsrc.DOS_00828=0;MCHP.modsrc.DOS_01116=0;MCHP.modsrc.DOS_01017_RPORx=0;MCHP.modsrc.DOS_01017_RPINRx=0;MCHP.modsrc.DOS_01555_nvm_tsmc18_v2_16bit=0;MCHP.modsrc.DOS_00804=0;MCHP.modsrc.DOS_00826=0;MCHP.modsrc.DOS_01555_TLAK_PMDx=0;MCHP.modsrc.DOS_01555_TLAK_INT_=0;MCHP.modsrc.DOS_00933=0;MCHP.modsrc.DOS_01555=0;MCHP.modsrc.DOS_01555_ptg=0;MCHP.modsrc.DOS_00958=0;MCHP.modsrc.DOS_01117_PORTx=0;MCHP.modsrc.DOS_00999=0;MCHP.modsrc.DOS_01041=0;MCHP.modsrc.DOS_00892=0;MCHP.modsrc.DOS_01287_TLAC_PMDx=0;MCHP.modsrc.DOS_01287_TLAC_INT_=0;MCHP.modsrc.DOS_01424=0;MCHP.modsrc.DOS_01332=0;MCHP.modsrc.DOS_01468_PMBA_current_source=0;MCHP.modsrc.DOS_02291_PGA=0;MCHP.modsrc.DOS_01467_Comparator=0;MCHP.modsrc.DOS_01498_TLAY=0;MCHP.modsrc.DOS_00993_PLL_120MHz=0;MCHP.modsrc.DOS_01332_ptg_pc_v1=0;MCHP.modsrc.DOS_00958_pwm_TLAY=0;MCHP.modsrc.TLAY_IOPorts=0;MCHP.modsrc.DOS_00929q=0;MCHP.modsrc.DOS_02415_spi_v5=0;MCHP.modsrc.DOS_RPINRx_16bit_2=0;MCHP.modsrc.DOS_01497_TLAH_PMDx=0;MCHP.modsrc.DOS_02550_TLAL_INT=0;MCHP.modsrc.DOS_00958_pwm_TLAH=0;MCHP.modsrc.DOS_01287_TLAH_INT_=0;MCHP.modsrc.DOS_01113=0;MCHP.modsrc.DOS_01017_PMDx=0;MCHP.modsrc.DOS_00927=0;MCHP.modsrc.DOS_01080=0;MCHP.modsrc.DOS_00794_cpu_16bit_v3=0;MCHP.modsrc.DOS_02192_TLCD_PMDx=0;MCHP.modsrc.DOS_02192_TLCD_INT_=0;MCHP.modsrc.DOS_02192_cmp=0;MCHP.modsrc.DOS_00958_pwm_TLCD=0;MCHP.modsrc.DOS_02192_PORTx_TLCD=0;MCHP.modsrc.DOS_00936=0;MCHP.modsrc.DOS_00995=0;MCHP.modsrc.DOS_00546=0;MCHP.modsrc.DOS_00474=0;MCHP.modsrc.DOS_02481_WACP_Config=0;MCHP.modsrc.DOS_03088_pfm_cache_ocp_v2_WACK=0;MCHP.modsrc.DOS_02819_pfm_ctrl_32bit_upb_v2=0;MCHP.modsrc.DOS_02674_wdt_upb_v1_32bit=0;MCHP.modsrc.DOS_01520_wdt_dmt_upb_v1=0;MCHP.modsrc.DOS_02869_icd_jtag_bvci_upb_v2=0;MCHP.modsrc.DOS_02823_WACJ_clk_cru_upb_v2=0;MCHP.modsrc.DOS_02823_WACN_clk_cru_upb_v2=0;MCHP.modsrc.DOS_01423_RPINRx=0;MCHP.modsrc.DOS_02481_RPORx=0;MCHP.modsrc.DOS_02511_pwr_sib_upb_v1_32bit=0;MCHP.modsrc.DOS_02907_WACP_int_evic_v3=0;MCHP.modsrc.DOS_01500_dma_bvci_v2=0;MCHP.modsrc.DOS_02141_tmr_classa_pb_v2=0;MCHP.modsrc.DOS_02815_tmr_classb_upb_v1=0;MCHP.modsrc.DOS_00740_icap_pb_v1=0;MCHP.modsrc.DOS_00749_ocmp_pb_v1=0;MCHP.modsrc.DOS_01441_i2c_upb_v1_32bit=0;MCHP.modsrc.DOS_01329_spi_pb_v2=0;MCHP.modsrc.DOS_02478_uart_irda_upb_v1_32bit=0;MCHP.modsrc.DOS_01477_pwm_mc_upb_v1=0;MCHP.modsrc.DOS_01494_qei_32b_upb_v1=0;MCHP.modsrc.DOS_03554_cmp_control_upb_v2_32bit=0;MCHP.modsrc.DOS_01445_dac_nbit__control_upb_v1_32bit=0;MCHP.modsrc.DOS_01461_afe_ctmu_con_upb_v1=0;MCHP.modsrc.DOS_01577_cla_clc_upb_v1_32bit=0;MCHP.modsrc.DOS_02467_gpio_ports_upb_v1=0;MCHP.modsrc.DOS_02508_WACP_adc_sar_ctrl_upb_v1=0;MCHP.modsrc.DOS_01261_tmr_rtcc_WACJ_K_N_P_pb_v2=0;MCHP.modsrc.DOS_EIP_00136_ssx_v1=0;MCHP.modsrc.DOS_02481_WACK_MC_Config=0;MCHP.modsrc.DOS_02907_WACN_GP_int_evic_v3=0;MCHP.modsrc.DOS_02508_adc_sar_ctrl_upb_v1_PIC32MK=0;MCHP.modsrc.DOS_01261_tmr_rtcc_pb_v2=0;MCHP.modsrc.DOS_01475_lpwr_deep_sleep_ctrl_v2=0;MCHP.modsrc.DOS_02907_WACN_MC_int_evic_v3=0;MCHP.modsrc.DOS_03247_can_fd_upb_v2_pic32mk=0;MCHP.modsrc.DOS_02907_WACK_MC_int_evic_v3=0;MCHP.modsrc.DOS_02514_dfm_strl_sst_upb_v1=0;MCHP.modsrc.DOS_02472_ppi_pmp16_upb_v1=0;MCHP.modsrc.DOS_02813a_usb_otgcore_pb_v3=0;MCHP.modsrc.DOS_02481_WACJ_MC_Config=0;MCHP.modsrc.DOS_02569_pfm_cache_ocp_v1=0;MCHP.modsrc.DOS_02481_WACJ_MC_int_evic_v3=0;MCHP.modsrc.DOS_01459_ptg_pc_upb_v1_SIC=0;MCHP.modsrc.DOS_01427_cmp_control_upb_v1_32bit=0;MCHP.modsrc.DOS_01152_can_bvci_v1=0;MCHP.modsrc.DOS_02787_WACD_Config=0;MCHP.modsrc.DOS_00800_dac_4bit_ctrl_pb_v1=0;MCHP.modsrc.DOS_01539_icd_jtag_pb_v2=0;MCHP.modsrc.DOS_02823_clk_cru_upb_v2=0;MCHP.modsrc.DOS_01423_RPORx=0;MCHP.modsrc.DOS_02907_WACD_int_evic_v3=0;MCHP.modsrc.DOS_00734_uart_irda_pb_v1=0;MCHP.modsrc.DOS_00687_tmr_classa_pb_v1=0;MCHP.modsrc.DOS_00745_tmr_classb_pb_v1=0;MCHP.modsrc.DOS_02508_adc_sar_ctrl_upb_v1=0;MCHP.modsrc.DOS_00866_cmp_control_pb_v2=0;MCHP.modsrc.DOS_01114_eth_bvci_v1=0;MCHP.modsrc.DOS_02831_usb_clk_rst_v2=0;MCHP.modsrc.DOS_01643_pfm_cache_ahb_v2=0;MCHP.modsrc.DOS_EIP_00206r5_sqi_v2=0;MCHP.modsrc.DOS_EIP_00124_usb_hs_otgcore_v1=0;MCHP.modsrc.DOS_EIP_00218_math_rng_ahbs_v2=0;MCHP.modsrc.DOS_EIP_00109_ebi_v1=0;MCHP.modsrc.DOS_EIP_00158_crypto_v1=0;MCHP.PortBase=16;MCHP.PortPrefixe='P';MCHP.clock.PBxDIV=-1;MCHP.clock.CLKx_INTDIV=reshape([-1 -1 -1 -1 0 1 0 0 0 -1 -1 0 0],1,13);MCHP.clock.CLKx_FRACDIV=reshape([-1 -1 -1 -1 0 256 0 0 0 -1 -1 0 0],1,13);  MCHP_CRC=18978666  BTMODE=Device is in Single Boot (legacy) mode  RES1=Not used  PLLSS=Not used  RES2=Not used  ALTCMPI=Not used  BOREN1=Not used  ALTRB6=Not used  RETCFG=Not used  DFMCY=Not used  BSS2=No Boot Segment  BSEN=No Boot Segment  CWRP=Configuration Segment may be written  CSS=No Protection (other than CWRP)  AIVTDIS=Disable Alternate Vector Table  BSLIM=Not used  WDTEN=Disable  BTSWP=BOOTSWP instruction is disabled  DBCC=No Cross Connection between DAC outputs  CTXT1=Not Assigned  CTXT2=Not Assigned  SEQNUM=Not used  nSEQNUM=Not used  BOREN0=Enabled  DMTIVT=Not used  DMTCNT=2^8 (256)  DMTEN=Dead Man Timer is Disabled and can be enabled by software  ON=Not used  USERID=Not used  RESERVED1=Not used  PGL1WAY=Allow only one reconfiguration  FPLLRNG=34-68 MHz Input  FPLLICLK=FRC is input to the System PLL  FPLLMULT=PLL Multiply by 128  UPLLFSEL=USB PLL input is 24 MHz  DMTINTV=Window/Interval value is 127/128 counter value  WDTSPGM=WDT stops during Flash programming  FDMTEN=Deadman Timer is disabled  TRCEN=Trace features in the CPU are enabled  BOOTISA=Boot code and Exception code is MIPS32  FECCCON=ECC and Dynamic ECC are disabled (ECCCON bits are writable)  EXTDDRSIZE=Not used  FSLEEP=Flash is powered down when the device is in Sleep mode  DBGPER=Allow CPU access to all permission regions  EJTAGBEN=Normal EJTAG functionality  TSEQ=Not used  CSEQ=Not used  RWDTPS=1:1048576  RCLKSEL=Always use LPRC  SWDTPS=1:1048576  DMTIVTL=Not used  DMTIVTH=Not used  DMTCNTL=Not used  DMTCNTH=Not used  DMTDIS=Dead Man Timer is Disabled and can be enabled by software  SMBEN=SMBus input threshold is enabled  SPI2PIN=SPI2 uses I/O remap (PPS) pins  CTXT3=Not Assigned  CTXT4=Not Assigned  MBXM0=Mailbox register configured for Main data read (Secondary to Main data transfer)  MBXM1=Mailbox register configured for Main data read (Secondary to Main data transfer)  MBXM2=Mailbox register configured for Main data read (Secondary to Main data transfer)  MBXM3=Mailbox register configured for Main data read (Secondary to Main data transfer)  MBXM4=Mailbox register configured for Main data read (Secondary to Main data transfer)  MBXM5=Mailbox register configured for Main data read (Secondary to Main data transfer)  MBXM6=Mailbox register configured for Main data read (Secondary to Main data transfer)  MBXM7=Mailbox register configured for Main data read (Secondary to Main data transfer)  MBXM8=Mailbox register configured for Main data read (Secondary to Main data transfer)  MBXM9=Mailbox register configured for Main data read (Secondary to Main data transfer)  MBXM10=Mailbox register configured for Main data read (Secondary to Main data transfer)  MBXM11=Mailbox register configured for Main data read (Secondary to Main data transfer)  MBXM12=Mailbox register configured for Main data read (Secondary to Main data transfer)  MBXM13=Mailbox register configured for Main data read (Secondary to Main data transfer)  MBXM14=Mailbox register configured for Main data read (Secondary to Main data transfer)  MBXM15=Mailbox register configured for Main data read (Secondary to Main data transfer)  MBXHSA=MSIxMBXD15 assigned to mailbox handshake protocol block A  MBXHSB=MSIxMBXD15 assigned to mailbox handshake protocol block B  MBXHSC=MSIxMBXD15 assigned to mailbox handshake protocol block C  MBXHSD=MSIxMBXD15 assigned to mailbox handshake protocol block D  MBXHSE=MSIxMBXD15 assigned to mailbox handshake protocol block E  MBXHSF=MSIxMBXD15 assigned to mailbox handshake protocol block F  MBXHSG=MSIxMBXD15 assigned to mailbox handshake protocol block G  MBXHSH=MSIxMBXD15 assigned to mailbox handshake protocol block H  HSAEN=Mailbox data flow control handshake protocol block disabled  HSBEN=Mailbox data flow control handshake protocol block disabled  HSCEN=Mailbox data flow control handshake protocol block disabled  HSDEN=Mailbox data flow control handshake protocol block disabled  HSEEN=Mailbox data flow control handshake protocol block disabled  HSFEN=Mailbox data flow control handshake protocol block disabled  HSGEN=Mailbox data flow control handshake protocol block disabled  HSHEN=Mailbox data flow control handshake protocol block disabled  CPRA0=Main core owns pin  CPRA1=Main core owns pin  CPRA2=Main core owns pin  CPRA3=Main core owns pin  CPRA4=Main core owns pin  CPRB0=Main core owns pin  CPRB1=Main core owns pin  CPRB2=Main core owns pin  CPRB3=Main core owns pin  CPRB4=Main core owns pin  CPRB5=Main core owns pin  CPRB6=Main core owns pin  CPRB7=Main core owns pin  CPRB8=Main core owns pin  CPRB9=Main core owns pin  CPRB10=Main core owns pin  CPRB11=Main core owns pin  CPRB12=Main core owns pin  CPRB13=Main core owns pin  CPRB14=Main core owns pin  CPRB15=Main core owns pin  CPRC0=Main core owns pin  CPRC1=Main core owns pin  CPRC2=Main core owns pin  CPRC3=Main core owns pin  CPRC4=Main core owns pin  CPRC5=Main core owns pin  CPRC6=Main core owns pin  CPRC7=Main core owns pin  CPRC8=Main core owns pin  CPRC9=Main core owns pin  CPRC10=Main core owns pin  CPRC11=Main core owns pin  CPRC12=Main core owns pin  CPRC13=Main core owns pin  CPRC14=Main core owns pin  CPRC15=Main core owns pin  CPRD0=Main core owns pin  CPRD1=Main core owns pin  CPRD2=Main core owns pin  CPRD3=Main core owns pin  CPRD4=Main core owns pin  CPRD5=Main core owns pin  CPRD6=Main core owns pin  CPRD7=Main core owns pin  CPRD8=Main core owns pin  CPRD9=Main core owns pin  CPRD10=Main core owns pin  CPRD11=Main core owns pin  CPRD12=Main core owns pin  CPRD13=Main core owns pin  CPRD14=Main core owns pin  CPRD15=Main core owns pin  CPRE0=Main core owns pin  CPRE1=Main core owns pin  CPRE2=Main core owns pin  CPRE3=Main core owns pin  CPRE4=Main core owns pin  CPRE5=Main core owns pin  CPRE6=Main core owns pin  CPRE7=Main core owns pin  CPRE8=Main core owns pin  CPRE9=Main core owns pin  CPRE10=Main core owns pin  CPRE11=Main core owns pin  CPRE12=Main core owns pin  CPRE13=Main core owns pin  CPRE14=Main core owns pin  CPRE15=Main core owns pin  S1FNOSC=Internal Fast RC (FRC) Oscillator with postscaler  S1IESO=Start up with FRC; then switch  S1OSCIOFNC=general purpose digital I/O pin  S1FCKSM=Both Clock switching and Fail-safe Clock Monitor are disabled  S1PLLKEN=S1PLLKEN_ON  S1RWDTPS=1:1048576  S1RCLKSEL=Always use LPRC  S1WINDIS=Watchdog Timer operates in Non-Window mode  S1WDTWIN=WDT Window is 25% of WDT period  S1SWDTPS=1:1048576  S1FWDTEN=use WDTCON.ON bit  S1ICS=Communicate on PGC1 and PGD1  S1DEBUG=Not used  S1ISOLAT=The Secondary can operate (in debug mode) even if the SLVEN bit in the MSI is zero  S1NOBTSWP=BOOTSWP instruction is disabled  S1ALTI2C1=I2C1 mapped to SDA1/SCL1 pins  S1SPI1PIN=Secondary SPI1 uses I/O remap (PPS) pins  S1SSRE=Secondary generated resets will reset the Secondary Enable Bit in the MSI module  S1MSRE=The Main software oriented RESET events (RESET Op-Code; Watchdog timeout; TRAP reset; illegalInstruction) will also cause the Secondary subsystem to reset  S1CTXT1=Not Assigned  S1CTXT2=Not Assigned  S1CTXT3=Not Assigned  S1CTXT4=Not Assigned  BORLVL=Not used  BSSO=Not used  MCA=Not used  MAXTEMP=Not used  CFGAN14=Not used  CFGAN15=Not used  S1IOL1WAY=Not used  S1BSSO=Not used  S1BACKBUG=Not used  BISTDIS=mBIST on reset feature disabled  NOBTSWP=BOOTSWP instruction is disabled  S1BISTDIS=Secondary BIST on reset feature disabled  S1DMTIVTL=Not used  S1DMTIVTH=Not used  S1DMTCNTL=Not used  S1DMTCNTH=Not used  S1DMTDIS=Secondary Dead Man Timer is Disabled and can be enabled by software  BSEQ=Not used  IBSEQ=Not used  SMB3EN=SMBus 3.0 input levels  FUSBIDIO2=USBID pin is controlled by the USB2 module  FVBUSIO2=VBUSON pin is controlled by the USB2 module  FUSBIDIO1=USBID pin is controlled by the USB1 module  FVBUSIO1=VBUSON pin is controlled by the USB1 module  VBATBOREN=Disable ZPBOR during VBAT Mode  FDSEN=Enable DSEN bit in DSCON  BORSEL=BOR trip voltage 2.1v (Non-OPAMP deviced operation)  POSCFGAIN=Gain is G3  POSCAGCDLY=Settling time = 25ms x AGCRNG  POSCAGCRNG=Range 1x  POSCAGC=Automatic Gain Control for Oscillator  FDBGWP=Not used
      settings: SourceProductName=MPLAB Device Blocks for Simulink
  Mosfet (3) + RGB LEDs (1 2 6) : MCHP_Blockset/PWM IO/PWM_HS_FEP  Priority=-2000  PWMx_MODSEL=Center Aligned  PWMx_CLKSEL=Use divider circuit  PWM_ClockResolution_DIVSEL_TXT=auto  PWM_ClockResolution_FSCL_TXT="Resol: 50(ns)  -  MaxPer: 3.28(ms)"  PWM_ClockResolution_NoScaling_TXT="Resol: 5(ns)  -  MaxPer: 328(us)"  MaxPeriod_s=1e-3  InitPeriode_s=1e-3  InitDutyCycleP_s=0  InitDutyCycleS_s=10e-6  InitPhase_s=-1  evalin_ws=PWM1max=MCHP_Fun.Hex2num('40D86A0000000000');PWM2max=MCHP_Fun.Hex2num('40D86A0000000000');PWM3max=MCHP_Fun.Hex2num('40D86A0000000000');PWM6max=MCHP_Fun.Hex2num('40D86A0000000000');  SampleTime=.001  S_INPUT=[-1]  S_INPUT_Size=[3]  S_OUTPUT=[]  S_OUTPUT_Size=[]  S_ListCustomDatatype=S.S_ListCustomDatatype={};  MCHP_USER_INTERRUPTS=0  MCHP_PORT={PWMH1 }{PWMH1}32:4:D2;{PWMH2 }{PWMH2}32:4:D0;{PWMH3 }{PWMH3}32:4:C3;{PWMH6 }{PWMH6}32:4:D9;  MCHP_MASTERLINK=PICOOZ_OL_ExtMode_Curiosity_dsPIC33AK512MPS512/Microchip Master  MCHP_CRC=4823485  PWMx_PMOD=Complementary  PWM1_HL=PWMxH output enabled  PWM1_swap=off  PWM1H_pol=off  PWM1L_pol=off  PWM2_HL=PWMxH output enabled  PWM2_swap=off  PWM2H_pol=off  PWM2L_pol=off  PWM3_HL=PWMxH output enabled  PWM3_swap=off  PWM3H_pol=off  PWM3L_pol=off  PWM4_HL=not used  PWM4_swap=off  PWM4H_pol=off  PWM4L_pol=off  PWM5_HL=not used  PWM5_swap=off  PWM5H_pol=off  PWM5L_pol=off  PWM6_HL=PWMxH output enabled  PWM6_swap=off  PWM6H_pol=off  PWM6L_pol=off  PWM7_HL=not used  PWM7_swap=off  PWM7H_pol=off  PWM7L_pol=off  PWM8_HL=not used  PWM8_swap=off  PWM8H_pol=off  PWM8L_pol=off  PWM9_HL=not used  PWM9_swap=off  PWM9H_pol=off  PWM9L_pol=off  PWM10_HL=not used  PWM10_swap=off  PWM10H_pol=off  PWM10L_pol=off  PWM11_HL=not used  PWM11_swap=off  PWM11H_pol=off  PWM11L_pol=off  PWM12_HL=not used  PWM12_swap=off  PWM12H_pol=off  PWM12L_pol=off  PWM1_ShowTrig=off  PWM1_Init_PGxTRIGABC_s=[0 -1 -1 ]  PWM1_ADTRxEN1=ADC Trigger 1  PWM1_ADTRxEN2=none  PWM1_ADTRxEN3=none  PWM2_ShowTrig=off  PWM2_Init_PGxTRIGABC_s=[-1 -1 -1]  PWM2_ADTRxEN1=none  PWM2_ADTRxEN2=none  PWM2_ADTRxEN3=none  PWM3_ShowTrig=on  PWM3_Init_PGxTRIGABC_s=[0 -1 -1]  PWM3_ADTRxEN1=ADC Trigger 1  PWM3_ADTRxEN2=none  PWM3_ADTRxEN3=none  PWM4_ShowTrig=off  PWM4_Init_PGxTRIGABC_s=[-1 -1 -1]  PWM4_ADTRxEN1=none  PWM4_ADTRxEN2=none  PWM4_ADTRxEN3=none  PWM5_ShowTrig=off  PWM5_Init_PGxTRIGABC_s=[-1 -1 -1]  PWM5_ADTRxEN1=none  PWM5_ADTRxEN2=none  PWM5_ADTRxEN3=none  PWM6_ShowTrig=off  PWM6_Init_PGxTRIGABC_s=[-1 -1 -1]  PWM6_ADTRxEN1=none  PWM6_ADTRxEN2=none  PWM6_ADTRxEN3=none  PWM7_ShowTrig=off  PWM7_Init_PGxTRIGABC_s=[-1 -1 -1]  PWM7_ADTRxEN1=none  PWM7_ADTRxEN2=none  PWM7_ADTRxEN3=none  PWM8_ShowTrig=off  PWM8_Init_PGxTRIGABC_s=[-1 -1 -1]  PWM8_ADTRxEN1=none  PWM8_ADTRxEN2=none  PWM8_ADTRxEN3=none  BlockInput_VectorScalar=Independant Scalar  BlockInput_Period=Not a block input  BlockInput_DutyCycle=a Floating Point input within range [-1 1]  BlockInput_PhaseShift=Not a block input  BlockInput_SEVTCMP=Not a block input  BlockInput_TRIGx=Not a block input  BlockInput_DeadTime=Not a block input  BlockOutput_FaultDisabled=off  BlockOutput_Fault=on  DTC=Positive dead time (ensure period of time with PWM_H and PWM_L disasserted)  FLTSRC1_DTCMP_TXT=<empty>  FLTSRC2_DTCMP_TXT=<empty>  FLTSRC3_DTCMP_TXT=<empty>  FLTSRC4_DTCMP_TXT=<empty>  FLTSRC5_DTCMP_TXT=<empty>  FLTSRC6_DTCMP_TXT=<empty>  FLTSRC7_DTCMP_TXT=<empty>  FLTSRC8_DTCMP_TXT=<empty>  FLTSRC9_DTCMP_TXT=<empty>  FLTSRC10_DTCMP_TXT=<empty>  FLTSRC11_DTCMP_TXT=<empty>  FLTSRC12_DTCMP_TXT=<empty>  DeadTime_s=2e-6  DeadTimeAlt_s=2e-6  DeadTimeComp_s=0  FLTMODx=Disabled  FLTSRCx_TXT=<empty>  FLTDATx=PWM H/L -> 11  CLMODx=Disabled  CLSRCx_TXT=<empty>  CLDATx=PWM H/L -> 00  FLTLEBENx=off  CLLEBENx=off  LeadEdgeBlkPer_s=5e-7  PHRx=off  PHFx=off  PLRx=off  PLFx=off
      settings: SourceProductName=MPLAB Device Blocks for Simulink
  Pot : MCHP_Blockset/Analog IO/ADC HS 12b dsPICA  ADCREF=ADC 1 and ADC 2  ADC1_refChannel=Not used  ADC2_refChannel=Not used  ADC3_refChannel=Not used  ADC4_refChannel=Not used  ADC5_refChannel=0 (highest priority)  CALRATE=once at startup  VREF_RNG=3.0V to 3.6V  BUFEN=off  info=0  SampleTime=0.01  MCHP_PORT={ADC1_seq0.0}{ADC1A2}15:2:A2;{ADC2_seq0.0}{ADC2B0}15:2:B0;{ADC1_seq1.0}{ADC1A2}15:2:A2;{ADC2_seq1.0}{ADC2B0}15:2:B0;{ADC1_seq2.0}{ADC1A2}15:2:A2;{ADC2_seq2.0}{ADC2B0}15:2:B0;{ADC1_seq3.0}{ADC1A2}15:2:A2;{ADC2_seq3.0}{ADC2B0}15:2:B0;{ADC1_seq4.0}{ADC1A2}15:2:A2;{ADC2_seq4.0}{ADC2B0}15:2:B0;{ADC1_seq5.0}{ADC1A2}15:2:A2;{ADC2_seq5.0}{ADC2B0}15:2:B0;{ADC1_seq0.0}{ADC1A2}15:2:A2;{ADC2_seq0.0}{ADC2B0}15:2:B0;{ADC1_seq1.0}{ADC1A2}15:2:A2;{ADC2_seq1.0}{ADC2B0}15:2:B0;{ADC1_seq2.0}{ADC1A2}15:2:A2;{ADC2_seq2.0}{ADC2B0}15:2:B0;{ADC1_seq3.0}{ADC1A2}15:2:A2;{ADC2_seq3.0}{ADC2B0}15:2:B0;{ADC1_seq4.0}{ADC1A2}15:2:A2;{ADC2_seq4.0}{ADC2B0}15:2:B0;{ADC1_seq5.0}{ADC1A2}15:2:A2;{ADC2_seq5.0}{ADC2B0}15:2:B0;  MCHP_MASTERLINK=PICOOZ_OL_ExtMode_Curiosity_dsPIC33AK512MPS512/Microchip Master  MCHP_CRC=33250715  ADC_Synchronisation=off  ADC_Trig_TXT=off  ADC_TrigTimeStep=off  TrigSource_seq0_TXT=after this block evaluation  SampleTime_seq0_Tad_TXT="8.5 Tad  = 106ns  -  Rin < 11 kOhm"  ADC1_seq0_TXT=AD1 AN0 / A2 / Pin[25]  ADC1_seq0_align=Left aligned  ADC1_seq0_overSampling=x1 (12 bits)  ADC2_seq0_TXT=AD2 AN0 / B0 / Pin[41]  ADC2_seq0_align=Right aligned  ADC2_seq0_overSampling=x1 (12 bits)  ADC3_seq0_TXT=AD3 AN5 / A0 / Pin[4]  ADC3_seq0_align=Left aligned  ADC3_seq0_overSampling=x256 (16 bits)  ADC4_seq0_TXT=AD4 AN0 / B4 / Pin[57]  ADC4_seq0_align=Left aligned  ADC4_seq0_overSampling=x1 (12 bits)  ADC5_seq0_TXT=AD5 AN0 / A7 / Pin[5]  ADC5_seq0_align=Left aligned  ADC5_seq0_overSampling=x256 (16 bits)  ADC1_seq0_1_TXT=Not Used  ADC1_seq0_1_align=Right aligned  ADC1_seq0_1_overSampling=x1 (12 bits)  ADC2_seq0_1_TXT=Not Used  ADC2_seq0_1_align=Right aligned  ADC2_seq0_1_overSampling=x1 (12 bits)  ADC3_seq0_1_TXT=Not Used  ADC3_seq0_1_align=Right aligned  ADC3_seq0_1_overSampling=x1 (12 bits)  ADC4_seq0_1_TXT=Not Used  ADC4_seq0_1_align=Right aligned  ADC4_seq0_1_overSampling=x1 (12 bits)  ADC5_seq0_1_TXT=Not Used  ADC5_seq0_1_align=Right aligned  ADC5_seq0_1_overSampling=x1 (12 bits)  ADC1_seq0_2_TXT=Not Used  ADC1_seq0_2_align=Right aligned  ADC1_seq0_2_overSampling=x1 (12 bits)  ADC2_seq0_2_TXT=Not Used  ADC2_seq0_2_align=Right aligned  ADC2_seq0_2_overSampling=x1 (12 bits)  ADC3_seq0_2_TXT=Not Used  ADC3_seq0_2_align=Right aligned  ADC3_seq0_2_overSampling=x1 (12 bits)  ADC4_seq0_2_TXT=Not Used  ADC4_seq0_2_align=Right aligned  ADC4_seq0_2_overSampling=x1 (12 bits)  ADC5_seq0_2_TXT=Not Used  ADC5_seq0_2_align=Right aligned  ADC5_seq0_2_overSampling=x1 (12 bits)  ADC1_seq0_3_TXT=Not Used  ADC1_seq0_3_align=Right aligned  ADC1_seq0_3_overSampling=x1 (12 bits)  ADC2_seq0_3_TXT=Not Used  ADC2_seq0_3_align=Right aligned  ADC2_seq0_3_overSampling=x1 (12 bits)  ADC3_seq0_3_TXT=Not Used  ADC3_seq0_3_align=Right aligned  ADC3_seq0_3_overSampling=x1 (12 bits)  ADC4_seq0_3_TXT=Not Used  ADC4_seq0_3_align=Right aligned  ADC4_seq0_3_overSampling=x1 (12 bits)  ADC5_seq0_3_TXT=Not Used  ADC5_seq0_3_align=Right aligned  ADC5_seq0_3_overSampling=x1 (12 bits)  ADC1_seq0_4_TXT=Not Used  ADC1_seq0_4_align=Right aligned  ADC1_seq0_4_overSampling=x1 (12 bits)  ADC2_seq0_4_TXT=Not Used  ADC2_seq0_4_align=Right aligned  ADC2_seq0_4_overSampling=x1 (12 bits)  ADC3_seq0_4_TXT=Not Used  ADC3_seq0_4_align=Right aligned  ADC3_seq0_4_overSampling=x1 (12 bits)  ADC4_seq0_4_TXT=Not Used  ADC4_seq0_4_align=Right aligned  ADC4_seq0_4_overSampling=x1 (12 bits)  ADC5_seq0_4_TXT=Not Used  ADC5_seq0_4_align=Right aligned  ADC5_seq0_4_overSampling=x1 (12 bits)  ADC1_seq0_5_TXT=Not Used  ADC1_seq0_5_align=Right aligned  ADC1_seq0_5_overSampling=x1 (12 bits)  ADC2_seq0_5_TXT=Not Used  ADC2_seq0_5_align=Right aligned  ADC2_seq0_5_overSampling=x1 (12 bits)  ADC3_seq0_5_TXT=Not Used  ADC3_seq0_5_align=Right aligned  ADC3_seq0_5_overSampling=x1 (12 bits)  ADC4_seq0_5_TXT=Not Used  ADC4_seq0_5_align=Right aligned  ADC4_seq0_5_overSampling=x1 (12 bits)  ADC5_seq0_5_TXT=Not Used  ADC5_seq0_5_align=Right aligned  ADC5_seq0_5_overSampling=x1 (12 bits)  ADC_TRG2_ACCBRST_seq0=Burst - not interruptible  ADC1_NINSEL_seq0_TXT=Vss - single ended (unsigned)  ADC2_NINSEL_seq0_TXT=Vss - single ended (unsigned)  ADC3_NINSEL_seq0_TXT=Vss - single ended (unsigned)  ADC4_NINSEL_seq0_TXT=Vss - single ended (unsigned)  ADC5_NINSEL_seq0_TXT=Vss - single ended (unsigned)  TrigTimeStep_seq0=on  info_seq0=0  TrigSource_seq1_TXT=PWM1 adc trig 1  SampleTime_seq1_Tad_TXT="4.5 Tad  = 56.2ns  -  Rin < 5.2 kOhm"  ADC1_seq1_TXT=AD1 AN0 / A2 / Pin[25]  ADC1_seq1_align=Left aligned  ADC1_seq1_overSampling=x1 (12 bits)  ADC2_seq1_TXT=AD2 AN0 / B0 / Pin[41]  ADC2_seq1_align=Right aligned  ADC2_seq1_overSampling=x1 (12 bits)  ADC3_seq1_TXT=Not Used  ADC3_seq1_align=Left aligned  ADC3_seq1_overSampling=x1 (12 bits)  ADC4_seq1_TXT=AD4 AN0 / B4 / Pin[57]  ADC4_seq1_align=Left aligned  ADC4_seq1_overSampling=x1 (12 bits)  ADC5_seq1_TXT=Not Used  ADC5_seq1_align=Left aligned  ADC5_seq1_overSampling=x1 (12 bits)  ADC1_seq1_1_TXT=Not Used  ADC1_seq1_1_align=Right aligned  ADC1_seq1_1_overSampling=x1 (12 bits)  ADC2_seq1_1_TXT=Not Used  ADC2_seq1_1_align=Right aligned  ADC2_seq1_1_overSampling=x1 (12 bits)  ADC3_seq1_1_TXT=Not Used  ADC3_seq1_1_align=Right aligned  ADC3_seq1_1_overSampling=x1 (12 bits)  ADC4_seq1_1_TXT=Not Used  ADC4_seq1_1_align=Right aligned  ADC4_seq1_1_overSampling=x1 (12 bits)  ADC5_seq1_1_TXT=Not Used  ADC5_seq1_1_align=Right aligned  ADC5_seq1_1_overSampling=x1 (12 bits)  ADC1_seq1_2_TXT=Not Used  ADC1_seq1_2_align=Right aligned  ADC1_seq1_2_overSampling=x1 (12 bits)  ADC2_seq1_2_TXT=Not Used  ADC2_seq1_2_align=Right aligned  ADC2_seq1_2_overSampling=x1 (12 bits)  ADC3_seq1_2_TXT=Not Used  ADC3_seq1_2_align=Right aligned  ADC3_seq1_2_overSampling=x1 (12 bits)  ADC4_seq1_2_TXT=Not Used  ADC4_seq1_2_align=Right aligned  ADC4_seq1_2_overSampling=x1 (12 bits)  ADC5_seq1_2_TXT=Not Used  ADC5_seq1_2_align=Right aligned  ADC5_seq1_2_overSampling=x1 (12 bits)  ADC1_seq1_3_TXT=Not Used  ADC1_seq1_3_align=Right aligned  ADC1_seq1_3_overSampling=x1 (12 bits)  ADC2_seq1_3_TXT=Not Used  ADC2_seq1_3_align=Right aligned  ADC2_seq1_3_overSampling=x1 (12 bits)  ADC3_seq1_3_TXT=Not Used  ADC3_seq1_3_align=Right aligned  ADC3_seq1_3_overSampling=x1 (12 bits)  ADC4_seq1_3_TXT=Not Used  ADC4_seq1_3_align=Right aligned  ADC4_seq1_3_overSampling=x1 (12 bits)  ADC5_seq1_3_TXT=Not Used  ADC5_seq1_3_align=Right aligned  ADC5_seq1_3_overSampling=x1 (12 bits)  ADC1_seq1_4_TXT=Not Used  ADC1_seq1_4_align=Right aligned  ADC1_seq1_4_overSampling=x1 (12 bits)  ADC2_seq1_4_TXT=Not Used  ADC2_seq1_4_align=Right aligned  ADC2_seq1_4_overSampling=x1 (12 bits)  ADC3_seq1_4_TXT=Not Used  ADC3_seq1_4_align=Right aligned  ADC3_seq1_4_overSampling=x1 (12 bits)  ADC4_seq1_4_TXT=Not Used  ADC4_seq1_4_align=Right aligned  ADC4_seq1_4_overSampling=x1 (12 bits)  ADC5_seq1_4_TXT=Not Used  ADC5_seq1_4_align=Right aligned  ADC5_seq1_4_overSampling=x1 (12 bits)  ADC1_seq1_5_TXT=Not Used  ADC1_seq1_5_align=Right aligned  ADC1_seq1_5_overSampling=x1 (12 bits)  ADC2_seq1_5_TXT=Not Used  ADC2_seq1_5_align=Right aligned  ADC2_seq1_5_overSampling=x1 (12 bits)  ADC3_seq1_5_TXT=Not Used  ADC3_seq1_5_align=Right aligned  ADC3_seq1_5_overSampling=x1 (12 bits)  ADC4_seq1_5_TXT=Not Used  ADC4_seq1_5_align=Right aligned  ADC4_seq1_5_overSampling=x1 (12 bits)  ADC5_seq1_5_TXT=Not Used  ADC5_seq1_5_align=Right aligned  ADC5_seq1_5_overSampling=x1 (12 bits)  ADC_TRG2_ACCBRST_seq1=Burst - not interruptible  ADC1_NINSEL_seq1_TXT=Vss - single ended (unsigned)  ADC2_NINSEL_seq1_TXT=Vss - single ended (unsigned)  ADC3_NINSEL_seq1_TXT=Vss - single ended (unsigned)  ADC4_NINSEL_seq1_TXT=Vss - single ended (unsigned)  ADC5_NINSEL_seq1_TXT=Vss - single ended (unsigned)  TrigTimeStep_seq1=off  info_seq1=0  TrigSource_seq2_TXT=PWM1 adc trig 1  SampleTime_seq2_Tad_TXT="4.5 Tad  = 56.2ns  -  Rin < 5.2 kOhm"  ADC1_seq2_TXT=AD1 AN0 / A2 / Pin[25]  ADC1_seq2_align=Left aligned  ADC1_seq2_overSampling=x1 (12 bits)  ADC2_seq2_TXT=AD2 AN0 / B0 / Pin[41]  ADC2_seq2_align=Right aligned  ADC2_seq2_overSampling=x1 (12 bits)  ADC3_seq2_TXT=Not Used  ADC3_seq2_align=Left aligned  ADC3_seq2_overSampling=x1 (12 bits)  ADC4_seq2_TXT=AD4 AN0 / B4 / Pin[57]  ADC4_seq2_align=Left aligned  ADC4_seq2_overSampling=x1 (12 bits)  ADC5_seq2_TXT=Not Used  ADC5_seq2_align=Left aligned  ADC5_seq2_overSampling=x1 (12 bits)  ADC1_seq2_1_TXT=Not Used  ADC1_seq2_1_align=Right aligned  ADC1_seq2_1_overSampling=x1 (12 bits)  ADC2_seq2_1_TXT=Not Used  ADC2_seq2_1_align=Right aligned  ADC2_seq2_1_overSampling=x1 (12 bits)  ADC3_seq2_1_TXT=Not Used  ADC3_seq2_1_align=Right aligned  ADC3_seq2_1_overSampling=x1 (12 bits)  ADC4_seq2_1_TXT=Not Used  ADC4_seq2_1_align=Right aligned  ADC4_seq2_1_overSampling=x1 (12 bits)  ADC5_seq2_1_TXT=Not Used  ADC5_seq2_1_align=Right aligned  ADC5_seq2_1_overSampling=x1 (12 bits)  ADC1_seq2_2_TXT=Not Used  ADC1_seq2_2_align=Right aligned  ADC1_seq2_2_overSampling=x1 (12 bits)  ADC2_seq2_2_TXT=Not Used  ADC2_seq2_2_align=Right aligned  ADC2_seq2_2_overSampling=x1 (12 bits)  ADC3_seq2_2_TXT=Not Used  ADC3_seq2_2_align=Right aligned  ADC3_seq2_2_overSampling=x1 (12 bits)  ADC4_seq2_2_TXT=Not Used  ADC4_seq2_2_align=Right aligned  ADC4_seq2_2_overSampling=x1 (12 bits)  ADC5_seq2_2_TXT=Not Used  ADC5_seq2_2_align=Right aligned  ADC5_seq2_2_overSampling=x1 (12 bits)  ADC1_seq2_3_TXT=Not Used  ADC1_seq2_3_align=Right aligned  ADC1_seq2_3_overSampling=x1 (12 bits)  ADC2_seq2_3_TXT=Not Used  ADC2_seq2_3_align=Right aligned  ADC2_seq2_3_overSampling=x1 (12 bits)  ADC3_seq2_3_TXT=Not Used  ADC3_seq2_3_align=Right aligned  ADC3_seq2_3_overSampling=x1 (12 bits)  ADC4_seq2_3_TXT=Not Used  ADC4_seq2_3_align=Right aligned  ADC4_seq2_3_overSampling=x1 (12 bits)  ADC5_seq2_3_TXT=Not Used  ADC5_seq2_3_align=Right aligned  ADC5_seq2_3_overSampling=x1 (12 bits)  ADC1_seq2_4_TXT=Not Used  ADC1_seq2_4_align=Right aligned  ADC1_seq2_4_overSampling=x1 (12 bits)  ADC2_seq2_4_TXT=Not Used  ADC2_seq2_4_align=Right aligned  ADC2_seq2_4_overSampling=x1 (12 bits)  ADC3_seq2_4_TXT=Not Used  ADC3_seq2_4_align=Right aligned  ADC3_seq2_4_overSampling=x1 (12 bits)  ADC4_seq2_4_TXT=Not Used  ADC4_seq2_4_align=Right aligned  ADC4_seq2_4_overSampling=x1 (12 bits)  ADC5_seq2_4_TXT=Not Used  ADC5_seq2_4_align=Right aligned  ADC5_seq2_4_overSampling=x1 (12 bits)  ADC1_seq2_5_TXT=Not Used  ADC1_seq2_5_align=Right aligned  ADC1_seq2_5_overSampling=x1 (12 bits)  ADC2_seq2_5_TXT=Not Used  ADC2_seq2_5_align=Right aligned  ADC2_seq2_5_overSampling=x1 (12 bits)  ADC3_seq2_5_TXT=Not Used  ADC3_seq2_5_align=Right aligned  ADC3_seq2_5_overSampling=x1 (12 bits)  ADC4_seq2_5_TXT=Not Used  ADC4_seq2_5_align=Right aligned  ADC4_seq2_5_overSampling=x1 (12 bits)  ADC5_seq2_5_TXT=Not Used  ADC5_seq2_5_align=Right aligned  ADC5_seq2_5_overSampling=x1 (12 bits)  ADC_TRG2_ACCBRST_seq2=Burst - not interruptible  ADC1_NINSEL_seq2_TXT=Vss - single ended (unsigned)  ADC2_NINSEL_seq2_TXT=Vss - single ended (unsigned)  ADC3_NINSEL_seq2_TXT=Vss - single ended (unsigned)  ADC4_NINSEL_seq2_TXT=Vss - single ended (unsigned)  ADC5_NINSEL_seq2_TXT=Vss - single ended (unsigned)  TrigTimeStep_seq2=off  info_seq2=0  TrigSource_seq3_TXT=PWM1 adc trig 1  SampleTime_seq3_Tad_TXT="4.5 Tad  = 56.2ns  -  Rin < 5.2 kOhm"  ADC1_seq3_TXT=AD1 AN0 / A2 / Pin[25]  ADC1_seq3_align=Left aligned  ADC1_seq3_overSampling=x1 (12 bits)  ADC2_seq3_TXT=AD2 AN0 / B0 / Pin[41]  ADC2_seq3_align=Right aligned  ADC2_seq3_overSampling=x1 (12 bits)  ADC3_seq3_TXT=Not Used  ADC3_seq3_align=Left aligned  ADC3_seq3_overSampling=x1 (12 bits)  ADC4_seq3_TXT=AD4 AN0 / B4 / Pin[57]  ADC4_seq3_align=Left aligned  ADC4_seq3_overSampling=x1 (12 bits)  ADC5_seq3_TXT=Not Used  ADC5_seq3_align=Left aligned  ADC5_seq3_overSampling=x1 (12 bits)  ADC1_seq3_1_TXT=Not Used  ADC1_seq3_1_align=Right aligned  ADC1_seq3_1_overSampling=x1 (12 bits)  ADC2_seq3_1_TXT=Not Used  ADC2_seq3_1_align=Right aligned  ADC2_seq3_1_overSampling=x1 (12 bits)  ADC3_seq3_1_TXT=Not Used  ADC3_seq3_1_align=Right aligned  ADC3_seq3_1_overSampling=x1 (12 bits)  ADC4_seq3_1_TXT=Not Used  ADC4_seq3_1_align=Right aligned  ADC4_seq3_1_overSampling=x1 (12 bits)  ADC5_seq3_1_TXT=Not Used  ADC5_seq3_1_align=Right aligned  ADC5_seq3_1_overSampling=x1 (12 bits)  ADC1_seq3_2_TXT=Not Used  ADC1_seq3_2_align=Right aligned  ADC1_seq3_2_overSampling=x1 (12 bits)  ADC2_seq3_2_TXT=Not Used  ADC2_seq3_2_align=Right aligned  ADC2_seq3_2_overSampling=x1 (12 bits)  ADC3_seq3_2_TXT=Not Used  ADC3_seq3_2_align=Right aligned  ADC3_seq3_2_overSampling=x1 (12 bits)  ADC4_seq3_2_TXT=Not Used  ADC4_seq3_2_align=Right aligned  ADC4_seq3_2_overSampling=x1 (12 bits)  ADC5_seq3_2_TXT=Not Used  ADC5_seq3_2_align=Right aligned  ADC5_seq3_2_overSampling=x1 (12 bits)  ADC1_seq3_3_TXT=Not Used  ADC1_seq3_3_align=Right aligned  ADC1_seq3_3_overSampling=x1 (12 bits)  ADC2_seq3_3_TXT=Not Used  ADC2_seq3_3_align=Right aligned  ADC2_seq3_3_overSampling=x1 (12 bits)  ADC3_seq3_3_TXT=Not Used  ADC3_seq3_3_align=Right aligned  ADC3_seq3_3_overSampling=x1 (12 bits)  ADC4_seq3_3_TXT=Not Used  ADC4_seq3_3_align=Right aligned  ADC4_seq3_3_overSampling=x1 (12 bits)  ADC5_seq3_3_TXT=Not Used  ADC5_seq3_3_align=Right aligned  ADC5_seq3_3_overSampling=x1 (12 bits)  ADC1_seq3_4_TXT=Not Used  ADC1_seq3_4_align=Right aligned  ADC1_seq3_4_overSampling=x1 (12 bits)  ADC2_seq3_4_TXT=Not Used  ADC2_seq3_4_align=Right aligned  ADC2_seq3_4_overSampling=x1 (12 bits)  ADC3_seq3_4_TXT=Not Used  ADC3_seq3_4_align=Right aligned  ADC3_seq3_4_overSampling=x1 (12 bits)  ADC4_seq3_4_TXT=Not Used  ADC4_seq3_4_align=Right aligned  ADC4_seq3_4_overSampling=x1 (12 bits)  ADC5_seq3_4_TXT=Not Used  ADC5_seq3_4_align=Right aligned  ADC5_seq3_4_overSampling=x1 (12 bits)  ADC1_seq3_5_TXT=Not Used  ADC1_seq3_5_align=Right aligned  ADC1_seq3_5_overSampling=x1 (12 bits)  ADC2_seq3_5_TXT=Not Used  ADC2_seq3_5_align=Right aligned  ADC2_seq3_5_overSampling=x1 (12 bits)  ADC3_seq3_5_TXT=Not Used  ADC3_seq3_5_align=Right aligned  ADC3_seq3_5_overSampling=x1 (12 bits)  ADC4_seq3_5_TXT=Not Used  ADC4_seq3_5_align=Right aligned  ADC4_seq3_5_overSampling=x1 (12 bits)  ADC5_seq3_5_TXT=Not Used  ADC5_seq3_5_align=Right aligned  ADC5_seq3_5_overSampling=x1 (12 bits)  ADC_TRG2_ACCBRST_seq3=Burst - not interruptible  ADC1_NINSEL_seq3_TXT=Vss - single ended (unsigned)  ADC2_NINSEL_seq3_TXT=Vss - single ended (unsigned)  ADC3_NINSEL_seq3_TXT=Vss - single ended (unsigned)  ADC4_NINSEL_seq3_TXT=Vss - single ended (unsigned)  ADC5_NINSEL_seq3_TXT=Vss - single ended (unsigned)  TrigTimeStep_seq3=off  info_seq3=0  TrigSource_seq4_TXT=PWM1 adc trig 1  SampleTime_seq4_Tad_TXT="4.5 Tad  = 56.2ns  -  Rin < 5.2 kOhm"  ADC1_seq4_TXT=AD1 AN0 / A2 / Pin[25]  ADC1_seq4_align=Left aligned  ADC1_seq4_overSampling=x1 (12 bits)  ADC2_seq4_TXT=AD2 AN0 / B0 / Pin[41]  ADC2_seq4_align=Right aligned  ADC2_seq4_overSampling=x1 (12 bits)  ADC3_seq4_TXT=Not Used  ADC3_seq4_align=Left aligned  ADC3_seq4_overSampling=x1 (12 bits)  ADC4_seq4_TXT=AD4 AN0 / B4 / Pin[57]  ADC4_seq4_align=Left aligned  ADC4_seq4_overSampling=x1 (12 bits)  ADC5_seq4_TXT=Not Used  ADC5_seq4_align=Left aligned  ADC5_seq4_overSampling=x1 (12 bits)  ADC1_seq4_1_TXT=Not Used  ADC1_seq4_1_align=Right aligned  ADC1_seq4_1_overSampling=x1 (12 bits)  ADC2_seq4_1_TXT=Not Used  ADC2_seq4_1_align=Right aligned  ADC2_seq4_1_overSampling=x1 (12 bits)  ADC3_seq4_1_TXT=Not Used  ADC3_seq4_1_align=Right aligned  ADC3_seq4_1_overSampling=x1 (12 bits)  ADC4_seq4_1_TXT=Not Used  ADC4_seq4_1_align=Right aligned  ADC4_seq4_1_overSampling=x1 (12 bits)  ADC5_seq4_1_TXT=Not Used  ADC5_seq4_1_align=Right aligned  ADC5_seq4_1_overSampling=x1 (12 bits)  ADC1_seq4_2_TXT=Not Used  ADC1_seq4_2_align=Right aligned  ADC1_seq4_2_overSampling=x1 (12 bits)  ADC2_seq4_2_TXT=Not Used  ADC2_seq4_2_align=Right aligned  ADC2_seq4_2_overSampling=x1 (12 bits)  ADC3_seq4_2_TXT=Not Used  ADC3_seq4_2_align=Right aligned  ADC3_seq4_2_overSampling=x1 (12 bits)  ADC4_seq4_2_TXT=Not Used  ADC4_seq4_2_align=Right aligned  ADC4_seq4_2_overSampling=x1 (12 bits)  ADC5_seq4_2_TXT=Not Used  ADC5_seq4_2_align=Right aligned  ADC5_seq4_2_overSampling=x1 (12 bits)  ADC1_seq4_3_TXT=Not Used  ADC1_seq4_3_align=Right aligned  ADC1_seq4_3_overSampling=x1 (12 bits)  ADC2_seq4_3_TXT=Not Used  ADC2_seq4_3_align=Right aligned  ADC2_seq4_3_overSampling=x1 (12 bits)  ADC3_seq4_3_TXT=Not Used  ADC3_seq4_3_align=Right aligned  ADC3_seq4_3_overSampling=x1 (12 bits)  ADC4_seq4_3_TXT=Not Used  ADC4_seq4_3_align=Right aligned  ADC4_seq4_3_overSampling=x1 (12 bits)  ADC5_seq4_3_TXT=Not Used  ADC5_seq4_3_align=Right aligned  ADC5_seq4_3_overSampling=x1 (12 bits)  ADC1_seq4_4_TXT=Not Used  ADC1_seq4_4_align=Right aligned  ADC1_seq4_4_overSampling=x1 (12 bits)  ADC2_seq4_4_TXT=Not Used  ADC2_seq4_4_align=Right aligned  ADC2_seq4_4_overSampling=x1 (12 bits)  ADC3_seq4_4_TXT=Not Used  ADC3_seq4_4_align=Right aligned  ADC3_seq4_4_overSampling=x1 (12 bits)  ADC4_seq4_4_TXT=Not Used  ADC4_seq4_4_align=Right aligned  ADC4_seq4_4_overSampling=x1 (12 bits)  ADC5_seq4_4_TXT=Not Used  ADC5_seq4_4_align=Right aligned  ADC5_seq4_4_overSampling=x1 (12 bits)  ADC1_seq4_5_TXT=Not Used  ADC1_seq4_5_align=Right aligned  ADC1_seq4_5_overSampling=x1 (12 bits)  ADC2_seq4_5_TXT=Not Used  ADC2_seq4_5_align=Right aligned  ADC2_seq4_5_overSampling=x1 (12 bits)  ADC3_seq4_5_TXT=Not Used  ADC3_seq4_5_align=Right aligned  ADC3_seq4_5_overSampling=x1 (12 bits)  ADC4_seq4_5_TXT=Not Used  ADC4_seq4_5_align=Right aligned  ADC4_seq4_5_overSampling=x1 (12 bits)  ADC5_seq4_5_TXT=Not Used  ADC5_seq4_5_align=Right aligned  ADC5_seq4_5_overSampling=x1 (12 bits)  ADC_TRG2_ACCBRST_seq4=Burst - not interruptible  ADC1_NINSEL_seq4_TXT=Vss - single ended (unsigned)  ADC2_NINSEL_seq4_TXT=Vss - single ended (unsigned)  ADC3_NINSEL_seq4_TXT=Vss - single ended (unsigned)  ADC4_NINSEL_seq4_TXT=Vss - single ended (unsigned)  ADC5_NINSEL_seq4_TXT=Vss - single ended (unsigned)  TrigTimeStep_seq4=off  info_seq4=0  TrigSource_seq5_TXT=PWM1 adc trig 1  SampleTime_seq5_Tad_TXT="4.5 Tad  = 56.2ns  -  Rin < 5.2 kOhm"  ADC1_seq5_TXT=AD1 AN0 / A2 / Pin[25]  ADC1_seq5_align=Left aligned  ADC1_seq5_overSampling=x1 (12 bits)  ADC2_seq5_TXT=AD2 AN0 / B0 / Pin[41]  ADC2_seq5_align=Right aligned  ADC2_seq5_overSampling=x1 (12 bits)  ADC3_seq5_TXT=Not Used  ADC3_seq5_align=Left aligned  ADC3_seq5_overSampling=x1 (12 bits)  ADC4_seq5_TXT=AD4 AN0 / B4 / Pin[57]  ADC4_seq5_align=Left aligned  ADC4_seq5_overSampling=x1 (12 bits)  ADC5_seq5_TXT=Not Used  ADC5_seq5_align=Left aligned  ADC5_seq5_overSampling=x1 (12 bits)  ADC1_seq5_1_TXT=Not Used  ADC1_seq5_1_align=Right aligned  ADC1_seq5_1_overSampling=x1 (12 bits)  ADC2_seq5_1_TXT=Not Used  ADC2_seq5_1_align=Right aligned  ADC2_seq5_1_overSampling=x1 (12 bits)  ADC3_seq5_1_TXT=Not Used  ADC3_seq5_1_align=Right aligned  ADC3_seq5_1_overSampling=x1 (12 bits)  ADC4_seq5_1_TXT=Not Used  ADC4_seq5_1_align=Right aligned  ADC4_seq5_1_overSampling=x1 (12 bits)  ADC5_seq5_1_TXT=Not Used  ADC5_seq5_1_align=Right aligned  ADC5_seq5_1_overSampling=x1 (12 bits)  ADC1_seq5_2_TXT=Not Used  ADC1_seq5_2_align=Right aligned  ADC1_seq5_2_overSampling=x1 (12 bits)  ADC2_seq5_2_TXT=Not Used  ADC2_seq5_2_align=Right aligned  ADC2_seq5_2_overSampling=x1 (12 bits)  ADC3_seq5_2_TXT=Not Used  ADC3_seq5_2_align=Right aligned  ADC3_seq5_2_overSampling=x1 (12 bits)  ADC4_seq5_2_TXT=Not Used  ADC4_seq5_2_align=Right aligned  ADC4_seq5_2_overSampling=x1 (12 bits)  ADC5_seq5_2_TXT=Not Used  ADC5_seq5_2_align=Right aligned  ADC5_seq5_2_overSampling=x1 (12 bits)  ADC1_seq5_3_TXT=Not Used  ADC1_seq5_3_align=Right aligned  ADC1_seq5_3_overSampling=x1 (12 bits)  ADC2_seq5_3_TXT=Not Used  ADC2_seq5_3_align=Right aligned  ADC2_seq5_3_overSampling=x1 (12 bits)  ADC3_seq5_3_TXT=Not Used  ADC3_seq5_3_align=Right aligned  ADC3_seq5_3_overSampling=x1 (12 bits)  ADC4_seq5_3_TXT=Not Used  ADC4_seq5_3_align=Right aligned  ADC4_seq5_3_overSampling=x1 (12 bits)  ADC5_seq5_3_TXT=Not Used  ADC5_seq5_3_align=Right aligned  ADC5_seq5_3_overSampling=x1 (12 bits)  ADC1_seq5_4_TXT=Not Used  ADC1_seq5_4_align=Right aligned  ADC1_seq5_4_overSampling=x1 (12 bits)  ADC2_seq5_4_TXT=Not Used  ADC2_seq5_4_align=Right aligned  ADC2_seq5_4_overSampling=x1 (12 bits)  ADC3_seq5_4_TXT=Not Used  ADC3_seq5_4_align=Right aligned  ADC3_seq5_4_overSampling=x1 (12 bits)  ADC4_seq5_4_TXT=Not Used  ADC4_seq5_4_align=Right aligned  ADC4_seq5_4_overSampling=x1 (12 bits)  ADC5_seq5_4_TXT=Not Used  ADC5_seq5_4_align=Right aligned  ADC5_seq5_4_overSampling=x1 (12 bits)  ADC1_seq5_5_TXT=Not Used  ADC1_seq5_5_align=Right aligned  ADC1_seq5_5_overSampling=x1 (12 bits)  ADC2_seq5_5_TXT=Not Used  ADC2_seq5_5_align=Right aligned  ADC2_seq5_5_overSampling=x1 (12 bits)  ADC3_seq5_5_TXT=Not Used  ADC3_seq5_5_align=Right aligned  ADC3_seq5_5_overSampling=x1 (12 bits)  ADC4_seq5_5_TXT=Not Used  ADC4_seq5_5_align=Right aligned  ADC4_seq5_5_overSampling=x1 (12 bits)  ADC5_seq5_5_TXT=Not Used  ADC5_seq5_5_align=Right aligned  ADC5_seq5_5_overSampling=x1 (12 bits)  ADC_TRG2_ACCBRST_seq5=Burst - not interruptible  ADC1_NINSEL_seq5_TXT=Vss - single ended (unsigned)  ADC2_NINSEL_seq5_TXT=Vss - single ended (unsigned)  ADC3_NINSEL_seq5_TXT=Vss - single ended (unsigned)  ADC4_NINSEL_seq5_TXT=Vss - single ended (unsigned)  ADC5_NINSEL_seq5_TXT=Vss - single ended (unsigned)  TrigTimeStep_seq5=off  info_seq5=0
      settings: SourceProductName=MPLAB Device Blocks for Simulink
  Rate Transition : RateTransition  Deterministic=off  OutPortSampleTimeOpt=Multiple of input port sample time  OutPortSampleTimeMultiple=5
  Scope : Scope  NumInputPorts=2
      settings: ActiveDisplayYMinimum=-1.2  ActiveDisplayYMaximum=0.8
  Slider Gain : simulink/Math Operations/Slider Gain  gain=0.350  low=0  high=1
  Slider Gain1 : simulink/Math Operations/Slider Gain  gain=0.280  low=-1  high=1
  Steps Large : Subsystem
  UART Configuration : MCHP_Blockset/BUS UART/UART Configuration  UART_REF=1  BAUD_Choice_TXT="460800         [+0.01%]"  BAUD_Choice_IR_TXT=[]  BAUD_Custom=115200  INT_PRIORITY=0  ALT_IO=on  PIN_RX_TXT=D10 / P59 / Pin[99]  PIN_RX_INPUT_MODE=Hi-impedance (default)  PIN_TX_TXT=H0 / P113 / Pin[97]  PIN_TX_OUTPUT_MODE=Push-Pull (default)  MCHP_PORT="{UART1  Rx}{U1RX}3:0:P59;{UART1  Tx}{U1TX}3:0:P113;"  MCHP_MASTERLINK=PICOOZ_OL_ExtMode_Curiosity_dsPIC33AK512MPS512/Microchip Master  MCHP_COM_ExtPil=on  TX_IMPLEMENTATION=Circular Buffer  TX_IMPLEMENTATION_default=Circular Buffer  TX_INT_PRIORITY=5  TX_INT_WHEN=is empty  TX_INT_WHEN_default=is empty & last char is sent  TX_CIRCULAR_SIZE=128  TX_DMA_CHANNEL="0   (Lowest Priority)"  TX_DMA_SIZE=[]  TX_TASK_PROTECTION=Delay tasks (default)  TX_INTERRUPT_PROTECTION=Do not send on conflict (default)  TX_INTERRUPT_PROTECTION_default=Do not send on conflict (default)  RX_IMPLEMENTATION=Circular Buffer  RX_IMPLEMENTATION_default=Circular Buffer  RX_INT_PRIORITY=5  RX_INT_WHEN=is 3/4 fulll (contains 3 data characters)  RX_CIRCULAR_SIZE=128  RX_DMA_CHANNEL=0  RX_DMA_SIZE=0  DuplexMode=Full duplex (default)  PIN_RX_Inv=off  PIN_TX_Inv=off  PIN_RXTX_Inv=off  ParityBit=No parity (default)  StopBit=1 stop bit (default)  IRDA=off  IdleTime_choice_TXT=None  IdleTime_custom=2/50  FlowControl=None  PIN_CTS_TXT=A0 / P1 / Pin[4]  PIN_CTS_INPUT_MODE=Hi-impedance (default)  PIN_RTS_TXT=A0 / P1 / Pin[4]  PIN_RTS_OUTPUT_MODE=Push-Pull (default)  PIN_DSR_TXT=A0 / P1 / Pin[4]  PIN_DSR_INPUT_MODE=Hi-impedance (default)  PIN_DTR_TXT=A0 / P1 / Pin[4]  PIN_DTR_OUTPUT_MODE=Push-Pull (default)  InitSequence_chkbox=off  BAUD_Choice_InitSeq_TXT="110         [+73.40%]"  BAUD_Choice_IR_InitSeq_TXT=0  BAUD_Custom_InitSeq=0  InitSequence='Hello World'
      settings: SourceProductName=MPLAB Device Blocks for Simulink
  wires:
  Chirp/1 -> Slider Gain/1
  BEMF/1 -> Buffer/1
  Median/1 -> Bitwise NOT/1  "BEMFn"
  Buffer/1 -> Median/1
  Rate Transition/1 -> Scope/1  "PWM Duty Cycle"
  Direct Lookup Table (n-D) Chenillard/1 -> LED [0-8]1/1
  Counter Limited/1 -> Direct Lookup Table (n-D) Chenillard/1
  Slider Gain/1 -> Manual Switch1/2
  Constant/1 -> Slider Gain1/1
  Slider Gain1/1 -> Manual Switch/2
  MCU Load/1 -> Gain/1
  Pot/1 -> Display/1
  Gain/1 -> MCU load in %/1  "MCU load"
  Manual Switch/1 -> Rate Transition/1, Mosfet (3) + RGB LEDs (1 2 6)/3, Mosfet (3) + RGB LEDs (1 2 6)/2, Mosfet (3) + RGB LEDs (1 2 6)/1, Mosfet (3) + RGB LEDs (1 2 6)/4
  Manual Switch1/1 -> Manual Switch/1
  Steps Large/1(Out1) -> Manual Switch1/1
  Bitwise NOT/1 -> Scope/2  "BEMF"
